simulink library "vmc"  (R2021b)
settings: Solver=VariableStepAuto  StartTime=0.0  StopTime=10.0  RelTol=1e-3
undefined symbols (not defined in the file or in its folder): AVMC_ACCDeltaTqIGain4OVRD_X_kph, AVMC_ACCDeltaTqIGain4OVRD_Y_mps2, AVMC_ACCDeltaTqIGain_X_kph, AVMC_ACCDeltaTqIGain_Y_mps2, AVMC_ACCDeltaTqPGain_X_kph, AVMC_ACCDeltaTqPGain_Y_kph, AVMC_ACCLongSteadyCtrl_X_kph, AVMC_ADSPosGFBDeltaTq_X_kph, AVMC_ADSPosGFBDeltaTq_Y_mps2, AVMC_AggressJerkPCT4AT_X_kph, AVMC_AggressJerkPCT_X_kph, AVMC_AggressLimitPCT4AT_X_kph, AVMC_AggressLimitPCT_X_kph, AVMC_CCLongSteadyCtrl_X_kph, AVMC_DISCDeltaTqIGain_X_kph, AVMC_DISCDeltaTqIGain_Y_mps2, AVMC_DISCDeltaTqPGain_X_kph, AVMC_DISCDeltaTqPGain_Y_kph, AVMC_ESCRegenOut_X_kph, AVMC_ESCRegenOut_Y_Deg, AVMC_ESCRegenOutEnSpd_X_Deg, AVMC_ISOAccLimit_X_mps, AVMC_ISODecLimit_X_mps, AVMC_ISOJerk_X_mps, AVMC_LatESCRegenOut_X_kph, AVMC_LatESCRegenOut_Y_Deg, AVMC_LongAccDeadZone_X_kph, AVMC_LongAccFiltTsforP2_X_Gps, AVMC_MCPresBaseTq_X_bar, AVMC_MSALongSteadyCtrl_X_kph, AVMC_MSAPedalOvrd_X_kph, AVMC_MSASpdBand_X_kph, AVMC_MSATqDownEndTq_X_kph, AVMC_MSATqDownTime_X_kph, AVMC_OPDDisSlideRate_X_Deg, AVMC_OVRD2ActSR2FCMCMD_X_mps2, AVMC_PedalTqRWhlRatio_X_Nm, AVMC_PedalTqRWhlRatio_Y_gps, AVMC_PedalTqRWhlSlipGain_X_rat, AVMC_PedalTqRWhlSlipGain_Y_kph, AVMC_PedalTqRWhSTRGGain_X_deg, AVMC_PedalTqRWhSTRGGain_Y_kph, AVMC_RDCDetectTime_X_kph, AVMC_RDCDetectTime_Y_pct, AVMC_RDCEnSlideRate_X_Deg, AVMC_RearWhlTqRatio_X_Nm, AVMC_RearWhlTqRatio_Y_gps, AVMC_RearWhlTqSlipGain_X_rat, AVMC_RearWhlTqSlipGain_Y_kph, AVMC_RearWhlTqSTRGGain_X_deg, AVMC_RearWhlTqSTRGGain_Y_kph, AVMC_ReqBrkJoinDecSR_X_mps2, AVMC_SoftJerkPCT_X_kph, AVMC_SoftLimitPCT_X_kph, AVMC_StESCYaw_X_kph, AVMC_StESCYaw_Y_Deg, AVMC_StESCYawCom_X_kph, AVMC_StESCYawCom_Y_Gps, AVMC_TMSpdBaseTq_X_rpm, AVMC_VehHoldDecCtrlTime2_X_kph ... (+405)
libraries: hcu_lib x105, simulink x75, tqr x1, simulink_extras x1
(part 2 of 14)

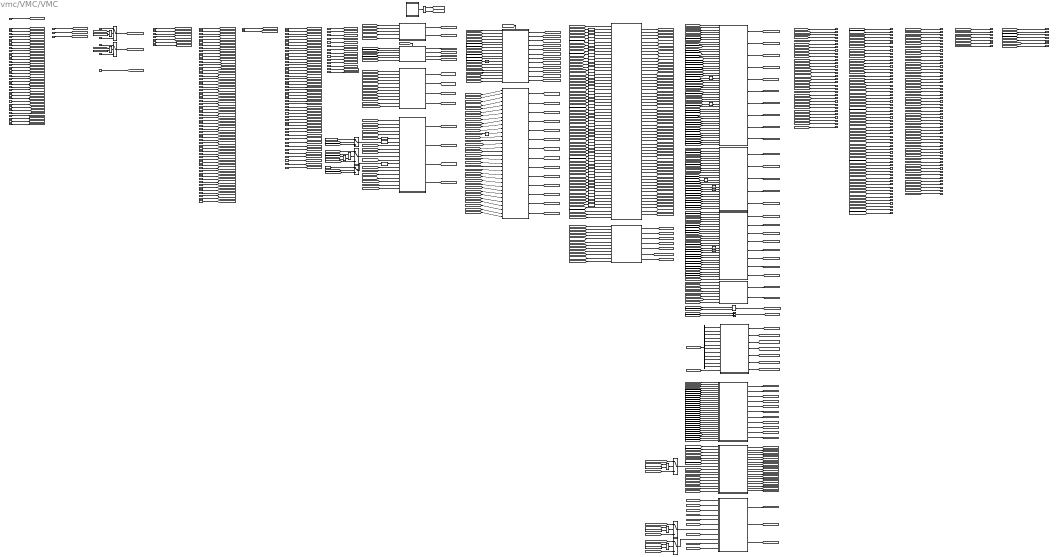
== system vmc/VMC/VMC ==
  note: AOICtrl
  note: VMC SW Version:
      | CR-No. B9 -> B10
      | Date: 2025/02/10
  note: Phase1_Add Functions for VCU
  note: FD
  note: GPIO
  note: CAN6
  note: DDM
  note: CAN3
  note: CAN2
  note: CAN1
  note: KPH2MPH_SetSpeed
  note: PreConditionCheck
  note: SPD2ACC
  note: VMC_FCM1
  note: SpeedArbitration
  note: ACC_CC_MSAWhlTq
  note: SafetyControl
  note: IMU
  note: SYS
  note: DSC
      | Test
      | Function
  note: For
      | DDM
      | 2024/12/21
  note: CAN4
  note: For
      | APS
      | 2025/02/07
  task_time_s : Inport
  VINP_DriverSeatBeltCmd_flg : Inport  Port=2
  VINP_MeterIndVehSpeed_kph : Inport  Port=3
  VINP_BrkSwSta_flg : Inport  Port=4
  VINP_EPBSta_enum : Inport  Port=5
  VINP_ACCAvail_flg : Inport  Port=6
  VINP_AEBAvail_flg : Inport  Port=7
  VINP_ESCOFFStatus_enum : Inport  Port=8
  VINP_VehSpeed_kph : Inport  Port=9
  VINP_LFRawWhlSpeed_kph : Inport  Port=10
  VINP_LFRawWhlSpeedV_flg : Inport  Port=11
  VINP_RFRawWhlSpeed_kph : Inport  Port=12
  VINP_RFRawWhlSpeedV_flg : Inport  Port=13
  VINP_LRRawWhlSpeed_kph : Inport  Port=14
  VINP_LRRawWhlSpeedV_flg : Inport  Port=15
  VINP_RRRawWhlSpeed_kph : Inport  Port=16
  VINP_RRRawWhlSpeedV_flg : Inport  Port=17
  VINP_LatAccel_Gps : Inport  Port=18
  VINP_LatAccelV_flg : Inport  Port=19
  VINP_GRADE_Deg : Inport  Port=20
  VINP_LongAccel_Gps : Inport  Port=21
  VINP_MCPressure_bar : Inport  Port=22
  VINP_ESCADASSta_enum : Inport  Port=23
  VINP_FrRBCActive_flg : Inport  Port=24
  VINP_RrRBCActive_flg : Inport  Port=25
  VINP_FrntAxlTrqReqBrk_Nm : Inport  Port=26
  VINP_RearAxlTrqReqBrk_Nm : Inport  Port=27
  VINP_BrkPedalPos_pct : Inport  Port=28
  VINP_SASAngle_Deg : Inport  Port=29
  VINP_ESCActive_flg : Inport  Port=30
  VINP_YawRate_degps : Inport  Port=31
  VINP_RDCActive_enum : Inport  Port=32
  VINP_LFWhlRotDir_enum : Inport  Port=33
  VINP_LRWhlRotDir_enum : Inport  Port=34
  VINP_RFWhlRotDir_enum : Inport  Port=35
  VINP_RRWhlRotDir_enum : Inport  Port=36
  VINP_Distanceunit_flg : Inport  Port=37
  VINP_IVISWCVibModeSta_enum : Inport  Port=38
  VINP_SmartEcoModeSW_flg : Inport  Port=39
  VINP_FrTMSpd_rpm : Inport  Port=40
  VINP_FrTMSpdNidec_rpm : Inport  Port=41
  VINP_RrTMSpd_rpm : Inport  Port=42
  VINP_RrTMSpdNidec_rpm : Inport  Port=43
  VINP_ADASAEBSta_enum : Inport  Port=44
  VINP_ADASACCSta_enum : Inport  Port=45
  VINP_ACCRequiredAccel_mps2 : Inport  Port=46
  VINP_ACCVehHoldReq_flg : Inport  Port=47
  VINP_ADASAEBReq_enum : Inport  Port=48
  VINP_ADASLKASta_enum : Inport  Port=49
  VINP_LKAStrToqReq_Nm : Inport  Port=50
  VINP_LKATOIFault_flg : Inport  Port=51
  VINP_LKATOIAct_enum : Inport  Port=52
  VINP_ADASFaultSta_flg : Inport  Port=53
  VINP_AEBVehHoldReq_flg : Inport  Port=54
  VINP_ADASDBSReq_enum : Inport  Port=55
  VINP_ACCObjDist_m : Inport  Port=56
  VINP_ACCObjRelSpd_mps : Inport  Port=57
  VINP_TimeGapLevel_enum : Inport  Port=58
  VINP_HazardWarningReq_flg : Inport  Port=59
  VINP_ADASForceIdle_flg : Inport  Port=60
  VINP_RightTurnLightReq_flg : Inport  Port=61
  VINP_LeftTurnLightReq_flg : Inport  Port=62
  VINP_ForceLowBeam_enum : Inport  Port=63
  VINP_ACCJerkUpperLimit_mps3 : Inport  Port=64
  VINP_ACCComfortBandUpper_mps2 : Inport  Port=65
  VINP_ACCJerkLowerLimit_mps3 : Inport  Port=66
  VINP_ACCComfortBandLower_mps2 : Inport  Port=67
  VINP_ADASVehSpdLim_raw32 : Inport  Port=68
  VINP_ADASShftPosnReqA_flg : Inport  Port=69
  VINP_ADASShftPosnReq_enum : Inport  Port=70
  VINP_ADASFCWSta_enum : Inport  Port=71
  VINP_ADASLDWSta_enum : Inport  Port=72
  VINP_ADASFltWrnReq_flg : Inport  Port=73
  VINP_ACCObjDstLvl_enum : Inport  Port=74
  VINP_ACCTakeoverReq_flg : Inport  Port=75
  VINP_ADASWarningMsg_enum : Inport  Port=76
  VINP_ADASCAMSpdLim_enum : Inport  Port=77
  VINP_TargetType_enum : Inport  Port=78
  VINP_ADASSLIFSpdLim_enum : Inport  Port=79
  VINP_LKAHODDisplayWarning_flg : Inport  Port=80
  VINP_LKAHODSoundWarning_flg : Inport  Port=81
  VINP_ADASLFCSta_enum : Inport  Port=82
  VINP_ADASLaneModeL_enum : Inport  Port=83
  VINP_ADASLaneModeR_enum : Inport  Port=84
  VINP_ADASSLIFSta_enum : Inport  Port=85
  VINP_ADASISASta_enum : Inport  Port=86
  VINP_ADASLDWMute_flg : Inport  Port=87
  VINP_ADASFCWMute_flg : Inport  Port=88
  VINP_ADASLFCHandsOffWarning_enum : Inport  Port=89
  VINP_LVDADisabled_flg : Inport  Port=90
  VINP_LVDAMuteSta_enum : Inport  Port=91
  VINP_LVDAFailinfo_flg : Inport  Port=92
  VINP_LVDAWarning_flg : Inport  Port=93
  VINP_LVDAACCStatusInformation_flg : Inport  Port=94
  VINP_ADASLFCWarnSound_enum : Inport  Port=95
  VINP_FCMACCmode_enum : Inport  Port=96
  VINP_ADASLanetypeR_enum : Inport  Port=97
  VINP_ADASLanetypeL_enum : Inport  Port=98
  VINP_ADASLanecurveL_raw32 : Inport  Port=99
  VINP_ADASLanecurveR_raw32 : Inport  Port=100
  VINP_ADASDrvInputTqBoostAct_flg : Inport  Port=101
  VINP_ADASStrWhlAngCtrlStatus_flg : Inport  Port=102
  VINP_ADASMaxAngCtrlOutTqLimit_Nm : Inport  Port=103
  VINP_ADASDrvInputTqBoostGain_pct : Inport  Port=104
  VINP_ADASAngCtrlTqWeightGain_pct : Inport  Port=105
  VINP_ADASDesStrWhlAngCtrlCmd_Deg : Inport  Port=106
  VINP_BrakeSWGPIO_flg : Inport  Port=107
  VINP_HoodSW_flg : Inport  Port=108
  APP_SpdLimit_flg : Inport  Port=109
  APP_SpdLimit : Inport  Port=110
  VINP_DIDGetDynoMode_flg : Inport  Port=111
  VINP_VehicleType_enum : Inport  Port=112
  VINP_SWCType_enum : Inport  Port=113
  VINP_APSStaSystem_enum : Inport  Port=114
  VINP_APSDecReqA_flg : Inport  Port=115
  VINP_APSDecReq_mps2 : Inport  Port=116
  VINP_APSReq_enum : Inport  Port=117
  VINP_APSShiftPosnReq_enum : Inport  Port=118
  VINP_APSSpeedCMD_kph : Inport  Port=119
  VINP_APSVMCReqA_flg : Inport  Port=120
  VINP_CAASVMCReqA_flg : Inport  Port=121
  VINP_APSVRqEPASCtrl_flg : Inport  Port=122
  VINP_APSRqEPASCtrl_flg : Inport  Port=123
  VINP_APSAngleTarget_Deg : Inport  Port=124
  VBCM_DrDoorSW_flg : Inport  Port=125
  VDSC_DISCTurn_flg : Inport  Port=126
  VDSC_DISCSta_enum : Inport  Port=127
  VDSC_DISCTargetSpd_kph : Inport  Port=128
  VDSC_TurningSpdMovingflat_kph : Inport  Port=129
  VDSC_AutoTurnMode_flg : Inport  Port=130
  VDSC_AccDecResp_flg : Inport  Port=131
  VDSC_PreACC_flg : Inport  Port=132
  VDSC_PreACC_mps2 : Inport  Port=133
  VTQD_DriverWhlTqDem_Nm : Inport  Port=134
  VTQD_CoordWhlTqDemFr_Nm : Inport  Port=135
  VTQD_CoordWhlTqDemRr_Nm : Inport  Port=136
  VTQD_GearActualPosn_enum : Inport  Port=137
  VTQD_ExternalTqAllow_flg : Inport  Port=138
  VTQD_LowIdleAccPedal_flg : Inport  Port=139
  VTQD_ExtShftAllow_flg : Inport  Port=140
  VTQD_FrEDUAvailBrkRgnTq_Nm : Inport  Port=141
  VTQD_RrEDUAvailBrkRgnTq_Nm : Inport  Port=142
  VTQD_APSStaSys_enum : Inport  Port=143
  VTQD_APSDecReqA_flg : Inport  Port=144
  VTQD_APSDecReq_mps2 : Inport  Port=145
  VTQD_APSReq_enum : Inport  Port=146
  VTQD_AfterAvailableTqDemFr_Nm : Inport  Port=147
  VTQD_AfterAvailableTqDemRr_Nm : Inport  Port=148
  VTQD_EquivAccPedalSWSta_flg : Inport  Port=149
  VTQD_ExtDoorAllow_flg : Inport  Port=150
  VTQD_SpdCtrlSta_flg : Inport  Port=151
  VTQD_SpdCtrlMode_enum : Inport  Port=152
  VTQD_RegenMode_enum : Inport  Port=153
  VTQD_SetSpd_kph : Inport  Port=154
  VTQD_SWC2ResUpSta_flg : Inport  Port=155
  VTQD_SWC2SetdownSta_flg : Inport  Port=156
  VTQD_SWC2CANCELSta_flg : Inport  Port=157
  VTQD_CreepBaseTqD_Nm : Inport  Port=158
  VTQD_VehActSpd_kph : Inport  Port=159
  VTQD_EVDriveMode_enum : Inport  Port=160
  VTQD_SWC1CANCELSta_flg : Inport  Port=161
  VTQD_SWC1ResUpSta_flg : Inport  Port=162
  VTQD_SWC1SetdownSta_flg : Inport  Port=163
  VTQD_EPBCarWashMode_flg : Inport  Port=164
  VTQR_RrTMTqReq_Nm : Inport  Port=165
  VTQR_FrTMTqReq_Nm : Inport  Port=166
  VDHP_ActAPSPosn_pct : Inport  Port=167
  <VPMM_DrivetrainSelect_enum> : Inport  Port=168
  BINP_IMU_outputs : Inport  Port=169  OutDataTypeStr=Bus: BINP_IMU_outputs
  VDDM_VMCLongCtrlProhibited_flg : Inport  Port=170
  VDDM_VMCLatCtrlProhibited_flg : Inport  Port=171
  VDDM_VMCESC1Err_flg : Inport  Port=172
  VDDM_VMCESC5Err_flg : Inport  Port=173
  VDDM_VMCEPSErr_flg : Inport  Port=174
  VDDM_VCURAPSErrLv2_flg : Inport  Port=175
  VDDM_VCURAPSErrLv3_flg : Inport  Port=176
  VINP_SCPSystemMode_enum : Inport  Port=177
  ACC_Function : Subsystem
  AND{4..6,9} (4 alike) : Logic  AllPortsSameDT=off  OutDataTypeStr=boolean
  APS function : Subsystem
  Add : Sum
  Bus Selector10 : BusSelector  OutputSignals=VINP_MemOffsetGyroX_raw16,VINP_MemOffsetGyroY_raw16,VINP_MemOffsetGyroZ_raw16,VINP_MemOffsetAccX_raw16,VINP_MemOffsetAccY_raw16,VINP_MemOffsetAccZ_raw16,VINP_SensingGyroX_raw16,VINP_SensingGyroY_raw16,VINP_SensingGyroZ_raw16,VINP_SensingAccX_raw16,VINP_SensingAccY_raw16,VINP_SensingAccZ_raw16
  Cast To Single{1,7,12,17,19..20,22,25..26,28..31,33..34,36,38..40,43..47,50,52,56..59,62} (31 alike) : DataTypeConversion  OutDataTypeStr=uint8
  Cast To Single{3..6,8..10,18,60..61} (10 alike) : DataTypeConversion  OutDataTypeStr=single
  Cast To Single{2,11,13..16,21,23..24,27,37,41..42,48..49,51,53..55} (19 alike) : DataTypeConversion  OutDataTypeStr=boolean
  Constant10 : Constant  Value=KVMC_RDCRzSource_flg
  Constant109 : Constant  Value=TRUE
  Constant11 : Constant  Value=KVMC_SlideRateGxSource_flg
  Constant14 : Constant  Value=ENUM_VEHICLETYPE_D31L24
  Constant15 : Constant  Value=ENUM_DISCSTA_ACTIVE
  Constant28 : Constant  Value=KVMC_RDCGySource_flg
  Constant6 : Constant  Value=ENUM_VEHICLETYPE_D31L24
  Constant7 : Constant  Value=ENUM_DISCSTA_ACTIVE
  CruiseControlFunction : Subsystem
  Equal1 : RelationalOperator  Operator=~=  OutDataTypeStr=boolean  RndMeth=Simplest
  Equal2 : RelationalOperator  Operator=~=  OutDataTypeStr=boolean  RndMeth=Simplest
  FeatureSetSpeed : Subsystem
  Function-Call Split : FunctionCallSplit  IconShape=distinctive  NumOutputPorts=2  OutputPortLayout=default
  IMU : Subsystem
  LFCAOIControl : Subsystem
  Logical Operator : Logic  Operator=OR  AllPortsSameDT=off  OutDataTypeStr=boolean
  Long Acceleration Calculation : Subsystem
  MSA function : Subsystem
  PreConditionCheck : Subsystem
  RDC Determination : Subsystem
  Relational Operator8 : RelationalOperator  Operator=~=  OutDataTypeStr=boolean  RndMeth=Simplest
  SPD2ACC : Subsystem
  SafetyControl : Subsystem  TreatAsAtomicUnit=on
  Scheduler : Stateflow chart  TreatAsAtomicUnit=on
  Slide Rate  Calculation : Subsystem
  SpeedArbitration : Subsystem
  SpeedCalculation : Subsystem  TreatAsAtomicUnit=on
  Switch{1..8} (8 alike) : Switch  Criteria=u2 > Threshold
  Unit Delay{,1..2,5..8} (7 alike) : UnitDelay  SampleTime=-1  HasFrameUpgradeWarning=on
  VMC_FCM1 : Subsystem
  initial = 0 : UnitDelay  SampleTime=-1  HasFrameUpgradeWarning=on
  VVMC_FeatSetSpdFinal_raw32 : Outport
  VVMC_VehicleSpeed_mph : Outport  Port=2
  VVMC_VehicleSpeed_kph : Outport  Port=3
  VVMC_MeterIndSpeed_raw32 : Outport  Port=4
  VVMC_MeterIndSpeedForCalcu_kph : Outport  Port=5
  VVMC_VMCAEBCtrlAvail_flg : Outport  Port=6
  VVMC_VMCACCCtrlAvail_flg : Outport  Port=7
  VVMC_VMCCCCtrlAvail_flg : Outport  Port=8
  VVMC_VMCMSACtrlAvail_flg : Outport  Port=9
  VVMC_FeatArbitrSta_enum : Outport  Port=10
  VVMC_FeatReqSpd_kph : Outport  Port=11
  VVMC_JerkPCT_pct : Outport  Port=12
  VVMC_LimitPCT_pct : Outport  Port=13
  VVMC_LFWhlSpeedRollAve_kph : Outport  Port=14
  VVMC_RFWhlSpeedRollAve_kph : Outport  Port=15
  VVMC_LRWhlSpeedRollAve_kph : Outport  Port=16
  VVMC_RRWhlSpeedRollAve_kph : Outport  Port=17
  VVMC_FrontRearSlipRatioCtrl_flg : Outport  Port=18
  VVMC_RearWhlSlipRatioCtrl_flg : Outport  Port=19
  VVMC_SingleWhlSlipRatioCtrl_flg : Outport  Port=20
  VVMC_LatAccCtrl_flg : Outport  Port=21
  VVMC_SafetyCtrl_flg : Outport  Port=22
  VVMC_EstSlope_Deg : Outport  Port=23
  VVMC_SPD2ACCAct_flg : Outport  Port=24
  VVMC_AccCalcuPID_mps2 : Outport  Port=25
  VVMC_ISOAccLimit_mps2 : Outport  Port=26
  VVMC_ISODecLimit_mps2 : Outport  Port=27
  VVMC_ISOJerkLimit_mps3 : Outport  Port=28
  VVMC_ACCRequiredAccel_mps2 : Outport  Port=29
  VVMC_DISCReqAcc_mps2 : Outport  Port=30
  VVMC_FeatArbitrFinal_enum : Outport  Port=31
  VVMC_ActACCRequiredAccel_mps2 : Outport  Port=32
  VVMC_LateralCtrl_flg : Outport  Port=33
  VVMC_ADASLKASta_enum : Outport  Port=34
  VVMC_LKAStrToqReq_Nm : Outport  Port=35
  VVMC_LKATOIFault_flg : Outport  Port=36
  VVMC_LKATOIAct_enum : Outport  Port=37
  VVMC_ADASAEBReq_enum : Outport  Port=38
  VVMC_ADASFaultSta_flg : Outport  Port=39
  VVMC_AEBVehHoldReq_flg : Outport  Port=40
  VVMC_ACCVehHoldReq_flg : Outport  Port=41
  VVMC_ADASDBSReq_enum : Outport  Port=42
  VVMC_ADASACCSta_enum : Outport  Port=43
  VVMC_ACCObjDist_m : Outport  Port=44
  VVMC_ACCObjRelSpd_mps : Outport  Port=45
  VVMC_TimeGapLevel_enum : Outport  Port=46
  VVMC_ACCJerkUpperLimit_mps3 : Outport  Port=47
  VVMC_ACCComfortBandUpper_mps2 : Outport  Port=48
  VVMC_ACCJerkLowerLimit_mps3 : Outport  Port=49
  VVMC_ACCComfortBandLower_mps2 : Outport  Port=50
  VVMC_ADASVehSpdLim_raw32 : Outport  Port=51
  VVMC_ADASShftPosnReqA_flg : Outport  Port=52
  VVMC_ADASShftPosnReq_enum : Outport  Port=53
  VVMC_ADASForceIdle_flg : Outport  Port=54
  VVMC_HazardWarningReq_flg : Outport  Port=55
  VVMC_RightTurnLightReq_flg : Outport  Port=56
  VVMC_LeftTurnLightReq_flg : Outport  Port=57
  VVMC_ADASFCWSta_enum : Outport  Port=58
  VVMC_ADASLDWSta_enum : Outport  Port=59
  VVMC_ADASFltWrnReq_flg : Outport  Port=60
  VVMC_ACCObjDstLvl_enum : Outport  Port=61
  VVMC_ForceLowBeam_enum : Outport  Port=62
  VVMC_ACCTakeoverReq_flg : Outport  Port=63
  VVMC_ADASWarningMsg_enum : Outport  Port=64
  VVMC_ADASCAMSpdLim_enum : Outport  Port=65
  VVMC_TargetType_enum : Outport  Port=66
  VVMC_ADASSLIFSpdLim_enum : Outport  Port=67
  VVMC_LKAHODDisplayWarning_flg : Outport  Port=68
  VVMC_LKAHODSoundWarning_flg : Outport  Port=69
  VVMC_ADASLFCSta_enum : Outport  Port=70
  VVMC_ADASLaneModeL_enum : Outport  Port=71
  VVMC_ADASLaneModeR_enum : Outport  Port=72
  VVMC_ADASSLIFSta_enum : Outport  Port=73
  VVMC_ADASISASta_enum : Outport  Port=74
  VVMC_ADASLDWMute_flg : Outport  Port=75
  VVMC_ADASFCWMute_flg : Outport  Port=76
  VVMC_ADASLFCHandsOffWarning_enum : Outport  Port=77
  VVMC_LVDADisabled_flg : Outport  Port=78
  VVMC_LVDAMuteSta_enum : Outport  Port=79
  VVMC_LVDAFailinfo_flg : Outport  Port=80
  VVMC_LVDAWarning_flg : Outport  Port=81
  VVMC_LVDAACCStatusInformation_flg : Outport  Port=82
  VVMC_ADASLFCWarnSound_enum : Outport  Port=83
  VVMC_FCMACCmode_enum : Outport  Port=84
  VVMC_ADASLanetypeR_enum : Outport  Port=85
  VVMC_ADASLanetypeL_enum : Outport  Port=86
  VVMC_ADASLanecurveL_raw32 : Outport  Port=87
  VVMC_ADASLanecurveR_raw32 : Outport  Port=88
  VVMC_ADASAEBSta_enum : Outport  Port=89
  VVMC_FCMLDWRequest_enum : Outport  Port=90
  VVMC_FCMLDWFault_flg : Outport  Port=91
  VVMC_ADASActive_flg : Outport  Port=92
  VVMC_ACCCtrlAvail_flg : Outport  Port=93
  VVMC_ADASNegReq_flg : Outport  Port=94
  VVMC_ACCPedalOvrd_flg : Outport  Port=95
  VVMC_ADASWhlTqReq_Nm : Outport  Port=96
  VVMC_AccPedalOvrdDISC_flg : Outport  Port=97
  VVMC_RearTqRatio_rat : Outport  Port=98
  VVMC_TimeGapCalcu_s : Outport  Port=99
  VVMC_CCCtrlSta_enum : Outport  Port=100
  VVMC_CruzActive_flg : Outport  Port=101
  VVMC_CCPedalOvrd_flg : Outport  Port=102
  VVMC_CruzWhlTqReq_Nm : Outport  Port=103
  VVMC_MSACtrlSta_enum : Outport  Port=104
  VVMC_MSAActive_flg : Outport  Port=105
  VVMC_MSAWhlTqReq_Nm : Outport  Port=106
  VVMC_APSCtrlAvail_flg : Outport  Port=107
  VVMC_APSActive_flg : Outport  Port=108
  VVMC_APSSpeedCMD_kph : Outport  Port=109
  VVMC_APSShiftPosnReq_enum : Outport  Port=110
  VVMC_APSStaSys_enum : Outport  Port=111
  VVMC_APSDecReqA_flg : Outport  Port=112
  VVMC_APSDecReq_mps2 : Outport  Port=113
  VVMC_APSReq_enum : Outport  Port=114
  VVMC_LongAcc_Gps : Outport  Port=115
  VVMC_RawWhlSpdSlideRate_pct : Outport  Port=116
  VVMC_LFWhlSpdSlideRate_pct : Outport  Port=117
  VVMC_RFWhlSpdSlideRate_pct : Outport  Port=118
  VVMC_LRWhlSpdSlideRate_pct : Outport  Port=119
  VVMC_RRWhlSpdSlideRate_pct : Outport  Port=120
  VVMC_PredictVehSpd_kph : Outport  Port=121
  VVMC_LF4WhlSpdSlideRate_pct : Outport  Port=122
  VVMC_RF4WhlSpdSlideRate_pct : Outport  Port=123
  VVMC_LR4WhlSpdSlideRate_pct : Outport  Port=124
  VVMC_RR4WhlSpdSlideRate_pct : Outport  Port=125
  VVMC_4WhlSpdSlideRate_pct : Outport  Port=126
  VVMC_ActMaxSlideRate_pct : Outport  Port=127
  VVMC_ActLFSlideRate_pct : Outport  Port=128
  VVMC_ActRFSlideRate_pct : Outport  Port=129
  VVMC_ActLRSlideRate_pct : Outport  Port=130
  VVMC_ActRRSlideRate_pct : Outport  Port=131
  VVMC_AltLWhlSlideRate_pct : Outport  Port=132
  VVMC_AltRWhlSlideRate_pct : Outport  Port=133
  VVMC_AltWhlSlideRate_pct : Outport  Port=134
  VVMC_CCMSASpdWar_flg : Outport  Port=135
  VVMC_IMUEnaCmd_flg : Outport  Port=136
  VVMC_RWDRDCActive_enum : Outport  Port=137
  VVMC_MSAWhlTqActive_flg : Outport  Port=138
  VVMC_RDCEnSlideRate_pct : Outport  Port=139
  VVMC_ActStESCYaw_Dps : Outport  Port=140
  VVMC_ACCOvrdMemTq_Nm : Outport  Port=141
  VVMC_CAASCtrlAvail_flg : Outport  Port=142
  VVMC_CAASActive_flg : Outport  Port=143
  "VVMC_ExtraMSACtrlSta_enum " : Outport  Port=144
  VVMC_CalibratedAccX_G : Outport  Port=145
  VVMC_CalibratedAccY_G : Outport  Port=146
  VVMC_CalibratedAccZ_G : Outport  Port=147
  VVMC_CalibratedGyroX_Dps : Outport  Port=148
  VVMC_CalibratedGyroY_Dps : Outport  Port=149
  VVMC_CalibratedGyroZ_Dps : Outport  Port=150
  VVMC_SetACCDisableAPS_flg : Outport  Port=151
  VVMC_FDCVMCAPSVRqEPSCtrl_flg : Outport  Port=152
  VVMC_FDCVMCAPSAngleTarget_deg : Outport  Port=153
  VVMC_FDCVMCAPSRqEPSCtrl_flg : Outport  Port=154
  VVMC_FDCVMCAngCtrlTqWtGn_pct : Outport  Port=155
  VVMC_FDCVMCDrInpTqBstAct_flg : Outport  Port=156
  VVMC_FDCVMCMaxAngCtrlOutTqLim_Nm : Outport  Port=157
  VVMC_FDCVMCDrInpTqBstGn_pct : Outport  Port=158
  wires:
  [VINP_VehSpeed_kph] -> SpeedArbitration/15(VINP_VehSpeed_kph)
  [VVMC_MeterIndSpeedForCalcu_kph] -> SpeedArbitration/14(VVMC_MeterIndSpeedForCalcu_kph)
  [VVMC_FeatArbitrFinal_enum] -> initial = 0/1
  [task_time_s] -> SPD2ACC/10(task_time_s)
  SpeedCalculation/4(VVMC_MeterIndSpeedForCalcu_kph) -> [VVMC_MeterIndSpeedForCalcu_kph]
  [VVMC_FeatReqSpd_kph] -> ACC_Function/19(VVMC_FeatReqSpd_kph)
  [task_time_s] -> PreConditionCheck/11(task_time_s)
  SpeedCalculation/3(VVMC_VehicleSpeed_kph) -> [VVMC_VehicleSpeed_kph]
  SpeedCalculation/2(VVMC_VehicleSpeed_mph) -> [VVMC_VehicleSpeed_mph]
  [VINP_VehSpeed_kph] -> Long Acceleration Calculation/3(VINP_VehSpeed_kph)
  [VINP_ESCADASSta_enum] -> ACC_Function/18(VINP_ESCADASSta_enum)  "VINP_ESCADASSta_enum"
  [VINP_MCPressure_bar] -> ACC_Function/17(VINP_MCPressure_bar)  "VINP_MCPressure_bar"
  [VINP_RrTMSpd_rpm] -> ACC_Function/16(VINP_RrTMSpd_rpm)  "VINP_RrTMSpd_rpm"
  [VINP_FrTMSpd_rpm] -> ACC_Function/15(VINP_FrTMSpd_rpm)  "VINP_FrTMSpd_rpm"
  VINP_FrRBCActive_flg/1 -> [VINP_FrRBCActive_flg]
  VINP_RrRBCActive_flg/1 -> [VINP_RrRBCActive_flg]
  VTQD_RegenMode_enum/1 -> [VTQD_RegenMode_enum]
  VINP_ESCADASSta_enum/1 -> [VINP_ESCADASSta_enum]
  VINP_MCPressure_bar/1 -> [VINP_MCPressure_bar]
  VINP_RrTMSpdNidec_rpm/1 -> Switch3/3
  [VINP_VehSpeed_kph] -> SPD2ACC/6(VINP_VehSpeed_kph)
  VINP_Distanceunit_flg/1 -> [VINP_Distanceunit_flg]
  [VINP_ADASACCSta_enum] -> SpeedArbitration/8(VINP_ADASACCSta_enum)  "VINP_ADASACCSta_enum"
  SPD2ACC/3(VVMC_FeatArbitrFinal_enum) -> [VVMC_FeatArbitrFinal_enum]
  [VINP_ACCObjDist_m] -> ACC_Function/12(VINP_ACCObjDist_m)  "VINP_ACCObjDist_m"
  ACC_Function/3(VVMC_ADASWhlTqReq_Nm) -> [VVMC_ADASWhlTqReq_Nm]
  [VTQD_CoordWhlTqDemFr_Nm] -> ACC_Function/4(VTQD_CoordWhlTqDemFr_Nm)  "VTQD_CoordWhlTqDemFr_Nm"
  [task_time_s] -> ACC_Function/1(task_time_s)  "task_time_s"
  SpeedArbitration/4(VVMC_LimitPCT_pct) -> [VVMC_LimitPCT_pct]
  [VTQD_ExternalTqAllow_flg] -> ACC_Function/3(VTQD_ExternalTqAllow_flg)  "VTQD_ExternalTqAllow_flg"
  [VINP_VehSpeed_kph] -> ACC_Function/7(VINP_VehSpeed_kph)
  SpeedArbitration/3(VVMC_JerkPCT_pct) -> [VVMC_JerkPCT_pct]
  [VVMC_VMCMSACtrlAvail_flg] -> SpeedArbitration/2(VVMC_VMCMSACtrlAvail_flg)
  [VINP_TimeGapLevel_enum] -> ACC_Function/14(VINP_TimeGapLevel_enum)  "VINP_TimeGapLevel_enum"
  [VVMC_FeatReqSpd_kph] -> SPD2ACC/3(VVMC_FeatReqSpd_kph)
  CruiseControlFunction/4(VVMC_CruzActive_flg) -> [VVMC_CruzActive_flg]
  CruiseControlFunction/2(VVMC_CCSpdWar_flg) -> [VVMC_CCSpdWar_flg]
  [VINP_LKATOIFault_flg] -> Cast To Single21/1
  [VTQD_SpdCtrlSta_flg] -> FeatureSetSpeed/2(VTQD_SpdCtrlSta_flg)  "VTQD_SpdCtrlSta_flg"
  Cast To Single20/1 -> VMC_FCM1/5(VINP_LKATOIAct_enum)  "VINP_LKATOIAct_enum"
  [VVMC_FeatSetSpdForCalcu_kph] -> CruiseControlFunction/12(VVMC_FeatSetSpdForCalcu_kph)
  [VVMC_MSACtrlSta_enum] -> SpeedArbitration/10(VVMC_MSACtrlSta_enum)  "VVMC_MSACtrlSta_enum"
  [VINP_DriverSeatBeltCmd_flg] -> PreConditionCheck/1(VINP_DriverSeatBeltCmd_flg)  "VINP_DriverSeatBeltCmd_flg"
  SpeedCalculation/1(VVMC_MeterIndSpeed_raw32) -> [VVMC_MeterIndSpeed_raw32]
  [VTQD_SetSpd_kph] -> FeatureSetSpeed/4(VTQD_SetSpd_kph)  "VTQD_SetSpd_kph"
  MSA function/3(VVMC_MSASpdWar_flg) -> [VVMC_MSASpdWar_flg]
  PreConditionCheck/4(VVMC_VMCMSACtrlAvail_flg) -> [VVMC_VMCMSACtrlAvail_flg]
  [VTQD_GearActualPosn_enum] -> PreConditionCheck/3(VTQD_GearActualPosn_enum)  "VTQD_GearActualPosn_enum"
  [VVMC_SafetyCtrl_flg] -> SPD2ACC/8(VVMC_SafetyCtrl_flg)  "VVMC_SafetyCtrl_flg"
  Cast To Single25/1 -> VMC_FCM1/10(VINP_ADASDBSReq_enum)  "VINP_ADASDBSReq_enum"
  CruiseControlFunction/1(VVMC_CCCtrlSta_enum) -> [VVMC_CCCtrlSta_enum]
  ACC_Function/1(VVMC_ACCCtrlAvail_flg) -> [VVMC_ACCCtrlAvail_flg]
  MSA function/4(VVMC_MSAActive_flg) -> [VVMC_MSAActive_flg]
  [VTQD_DriverWhlTqDem_Nm] -> MSA function/2(VTQD_DriverWhlTqDem_Nm)  "VTQD_DriverWhlTqDem_Nm"
  Logical Operator/1 -> [VVMC_CCMSASpdWar_flg]  "VVMC_CCMSASpdWar_flg"
  [VVMC_ActACCRequiredAccel_mps2] -> ACC_Function/10(VVMC_ActACCRequiredAccel_mps2)
  [VVMC_LongAcc_Gps] -> CruiseControlFunction/11(VVMC_LongAcc_Gps)
  ACC_Function/4(VVMC_ADASActive_flg) -> [VVMC_ADASActive_flg]
  [VINP_ADASAEBSta_enum] -> Cast To Single33/1
  [VTQD_ExternalTqAllow_flg] -> PreConditionCheck/9(VTQD_ExternalTqAllow_flg)  "VTQD_ExternalTqAllow_flg"
  [APP_SpdLimit_flg] -> FeatureSetSpeed/1(APP_SpdLimit_flg)  "APP_SpdLimit_flg"
  [VINP_APSStaSystem_enum] -> PreConditionCheck/8(VINP_APSStaSystem_enum)  "VINP_APSStaSystem_enum"
  PreConditionCheck/2(VVMC_VMCAEBCtrlAvail_flg) -> [VVMC_VMCAEBCtrlAvail_flg]
  FeatureSetSpeed/1(VVMC_FeatSetSpdFinal_raw32) -> [VVMC_FeatSetSpdFinal_raw32]
  [VINP_ACCAvail_flg] -> PreConditionCheck/5(VINP_ACCAvail_flg)  "VINP_ACCAvail_flg"
  SPD2ACC/1(VVMC_ACCRequiredAccel_mps2) -> [VVMC_ACCRequiredAccel_mps2]
  [VTQD_SpdCtrlMode_enum] -> CruiseControlFunction/4(<VTQD_SpdCtrlMode_enum>)  "VTQD_SpdCtrlMode_enum"
  [VVMC_MeterIndSpeedForCalcu_kph] -> SPD2ACC/7(VVMC_MeterIndSpeedForCalcu_kph)
  [VINP_ADASACCSta_enum] -> SPD2ACC/2(VINP_ADASACCSta_enum)  "VINP_ADASACCSta_enum"
  [VINP_ACCRequiredAccel_mps2] -> SPD2ACC/9(VINP_ACCRequiredAccel_mps2)  "VINP_ACCRequiredAccel_mps2"
  SPD2ACC/2(VVMC_DISCReqAcc_mps2) -> [VVMC_DISCReqAcc_mps2]  "VVMC_DISCReqAcc_mps2"
  [VDSC_DISCSta_enum] -> Switch4/3
  Cast To Single22/1 -> VMC_FCM1/6(VINP_ADASAEBReq_enum)  "VINP_ADASAEBReq_enum"
  [VINP_ACCVehHoldReq_flg] -> Cast To Single2/1
  [VVMC_FeatArbitrSta_enum] -> SPD2ACC/1(VVMC_FeatArbitrSta_enum)
  [VINP_LKATOIAct_enum] -> Cast To Single20/1
  Cast To Single24/1 -> VMC_FCM1/8(VINP_AEBVehHoldReq_flg)  "VINP_AEBVehHoldReq_flg"
  [VINP_AEBVehHoldReq_flg] -> Cast To Single24/1
  Cast To Single18/1 -> VMC_FCM1/3(VINP_LKAStrToqReq_Nm)  "VINP_LKAStrToqReq_Nm"
  [VINP_ADASDBSReq_enum] -> Cast To Single25/1
  [VINP_ADASLKASta_enum] -> Cast To Single19/1
  [VVMC_FeatArbitrFinal_enum] -> VMC_FCM1/1(VVMC_FeatArbitrFinal_enum)
  [VINP_ADASFaultSta_flg] -> Cast To Single23/1
  [VTQD_DriverWhlTqDem_Nm] -> ACC_Function/2(VTQD_DriverWhlTqDem_Nm)  "VTQD_DriverWhlTqDem_Nm"
  [VVMC_FeatSetSpdForCalcu_kph] -> SpeedArbitration/12(VVMC_FeatSetSpdForCalcu_kph)
  Cast To Single28/1 -> VMC_FCM1/11(VINP_ADASACCSta_enum)  "VINP_ADASACCSta_enum"
  [VINP_EPBSta_enum] -> PreConditionCheck/4(VINP_EPBSta_enum)  "VINP_EPBSta_enum"
  SpeedArbitration/1(VVMC_FeatArbitrSta_enum) -> [VVMC_FeatArbitrSta_enum]
  [VTQD_LowIdleAccPedal_flg] -> ACC_Function/6(VTQD_LowIdleAccPedal_flg)  "VTQD_LowIdleAccPedal_flg"
  [VVMC_MSASpdWar_flg] -> Logical Operator/2
  [VINP_LKAStrToqReq_Nm] -> Cast To Single18/1
  Long Acceleration Calculation/1(VVMC_LongAcc_Gps) -> [VVMC_LongAcc_Gps]
  CruiseControlFunction/3(VVMC_CruzWhlTqReq_Nm) -> [VVMC_CruzWhlTqReq_Nm]
  [VTQD_ExternalTqAllow_flg] -> MSA function/1(VTQD_ExternalTqAllow_flg)  "VTQD_ExternalTqAllow_flg"
  [VINP_BrkSwSta_flg] -> CruiseControlFunction/9(VINP_BrkSwSta_flg)  "VINP_BrkSwSta_flg"
  Cast To Single23/1 -> VMC_FCM1/7(VINP_ADASFaultSta_flg)  "VINP_ADASFaultSta_flg"
  [VINP_VehSpeed_kph] -> MSA function/5(VINP_VehSpeed_kph)
  PreConditionCheck/1(VVMC_VMCACCCtrlAvail_flg) -> [VVMC_VMCACCCtrlAvail_flg]
  [VINP_BrakeSWGPIO_flg] -> CruiseControlFunction/8(VINP_BrakeSWGPIO_flg)  "VINP_BrakeSWGPIO_flg"
  [VTQD_SWC1CANCELSta_flg] -> CruiseControlFunction/7(VTQD_SWC1CANCELSta_flg)  "VTQD_SWC1CANCELSta_flg"
  Cast To Single33/1 -> SpeedArbitration/6(VINP_ADASAEBSta_enum)  "VINP_ADASAEBSta_enum"
  Cast To Single34/1 -> SpeedArbitration/13(VDSC_DISCTurn_flg)  "VDSC_DISCTurn_flg"
  [VINP_GRADE_Deg] -> Long Acceleration Calculation/1(VINP_GRADE_Deg)  "VINP_GRADE_Deg"
  [VTQD_CoordWhlTqDemRr_Nm] -> ACC_Function/5(VTQD_CoordWhlTqDemRr_Nm)  "VTQD_CoordWhlTqDemRr_Nm"
  Cast To Single7/1 -> CruiseControlFunction/14(VINP_ADASAEBSta_enum)  "VINP_ADASAEBSta_enum"
  [VINP_ADASAEBReq_enum] -> SpeedArbitration/5(VINP_ADASAEBReq_enum)  "VINP_ADASAEBReq_enum"
  ACC_Function/5(VVMC_TimeGapCalcu_s) -> [VVMC_TimeGapCalcu_s]
  [VBCM_DrDoorSW_flg] -> PreConditionCheck/2(VBCM_DrDoorSW_flg)  "VBCM_DrDoorSW_flg"
  [VVMC_LongAcc_Gps] -> ACC_Function/8(VVMC_LongAcc_Gps)
  [VINP_AEBAvail_flg] -> PreConditionCheck/6(VINP_AEBAvail_flg)  "VINP_AEBAvail_flg"
  [VTQD_SpdCtrlMode_enum] -> MSA function/3(<VTQD_SpdCtrlMode_enum>)  "VTQD_SpdCtrlMode_enum"
  [VINP_ADASAEBSta_enum] -> Cast To Single7/1
  [VINP_VehSpeed_kph] -> CruiseControlFunction/10(VINP_VehSpeed_kph)
  [VVMC_FeatArbitrFinal_enum] -> CruiseControlFunction/13(VVMC_FeatArbitrFinal_enum)
  SpeedArbitration/2(VVMC_FeatReqSpd_kph) -> [VVMC_FeatReqSpd_kph]
  [VVMC_LimitPCT_pct] -> SPD2ACC/4(VVMC_LimitPCT_pct)
  [VVMC_VMCCCCtrlAvail_flg] -> SpeedArbitration/1(VVMC_VMCCCCtrlAvail_flg)
  [VTQD_SWC1SetdownSta_flg] -> CruiseControlFunction/6(VTQD_SWC1SetdownSta_flg)  "VTQD_SWC1SetdownSta_flg"
  [VTQD_SWC2SetdownSta_flg] -> MSA function/10(VTQD_SWC2SetdownSta_flg)  "VTQD_SWC2SetdownSta_flg"
  [VINP_ADASACCSta_enum] -> Cast To Single28/1
  Cast To Single2/1 -> VMC_FCM1/9(VINP_ACCVehHoldReq_flg)  "VINP_ACCVehHoldReq_flg"
  Cast To Single31/1 -> SpeedArbitration/7(VDSC_DISCSta_enum)  "VDSC_DISCSta_enum"
  [VINP_LongAccel_Gps] -> Long Acceleration Calculation/2(VINP_LongAccel_Gps)  "VINP_LongAccel_Gps"
  [APP_SpdLimit] -> FeatureSetSpeed/3(APP_SpdLimit)  "APP_SpdLimit"
  [VINP_ESCOFFStatus_enum] -> PreConditionCheck/7(VINP_ESCOFFStatus_enum)  "VINP_ESCOFFStatus_enum"
  [VTQD_SWC2ResUpSta_flg] -> MSA function/9(VTQD_SWC2ResUpSta_flg)  "VTQD_SWC2ResUpSta_flg"
  [VVMC_FeatSetSpdForCalcu_kph] -> ACC_Function/11(VVMC_FeatSetSpdForCalcu_kph)
  [VVMC_MeterIndSpeedForCalcu_kph] -> ACC_Function/13(VVMC_MeterIndSpeedForCalcu_kph)
  SPD2ACC/8(VVMC_ISOJerkLimit_mps3) -> [VVMC_ISOJerkLimit_mps3]
  SPD2ACC/4(VVMC_SPD2ACCAct_flg) -> [VVMC_SPD2ACCAct_flg]
  Cast To Single21/1 -> VMC_FCM1/4(VINP_LKATOIFault_flg)  "VINP_LKATOIFault_flg"
  ACC_Function/2(VVMC_ACCPedalOvrd_flg) -> [VVMC_ACCPedalOvrd_flg]
  MSA function/1(VVMC_MSACtrlSta_enum) -> [VVMC_MSACtrlSta_enum]
  [VVMC_FeatArbitrFinal_enum] -> MSA function/8(VVMC_FeatArbitrFinal_enum)
  [VVMC_LongAcc_Gps] -> MSA function/6(VVMC_LongAcc_Gps)
  [VTQD_SWC1ResUpSta_flg] -> CruiseControlFunction/5(VTQD_SWC1ResUpSta_flg)  "VTQD_SWC1ResUpSta_flg"
  [VTQD_DriverWhlTqDem_Nm] -> CruiseControlFunction/2(VTQD_DriverWhlTqDem_Nm)  "VTQD_DriverWhlTqDem_Nm"
  [VINP_ADASAEBReq_enum] -> Cast To Single22/1
  Switch2/1 -> SpeedArbitration/11(VDSC_DISCTargetSpd_kph)  "VDSC_DISCTargetSpd_kph"
  [VVMC_FeatSetSpdForCalcu_kph] -> MSA function/7(VVMC_FeatSetSpdForCalcu_kph)
  [VVMC_CCSpdWar_flg] -> Logical Operator/1
  [VTQD_ExternalTqAllow_flg] -> CruiseControlFunction/1(VTQD_ExternalTqAllow_flg)  "VTQD_ExternalTqAllow_flg"
  Cast To Single19/1 -> VMC_FCM1/2(VINP_ADASLKASta_enum)  "VINP_ADASLKASta_enum"
  [VTQD_LowIdleAccPedal_flg] -> CruiseControlFunction/3(VTQD_LowIdleAccPedal_flg)  "VTQD_LowIdleAccPedal_flg"
  PreConditionCheck/3(VVMC_VMCCCCtrlAvail_flg) -> [VVMC_VMCCCCtrlAvail_flg]
  SPD2ACC/7(VVMC_ISODecLimit_mps2) -> [VVMC_ISODecLimit_mps2]
  [VVMC_JerkPCT_pct] -> SPD2ACC/5(VVMC_JerkPCT_pct)
  [VVMC_ACCCtrlAvail_flg] -> PreConditionCheck/10(VVMC_ACCCtrlAvail_flg)  "VVMC_ACCCtrlAvail_flg"
  [VVMC_VMCAEBCtrlAvail_flg] -> SpeedArbitration/4(VVMC_VMCAEBCtrlAvail_flg)
  MSA function/2(VVMC_MSAWhlTqReq_Nm) -> [VVMC_MSAWhlTqReq_Nm]
  [VTQD_SWC2CANCELSta_flg] -> MSA function/4(VTQD_SWC2CANCELSta_flg)  "VTQD_SWC2CANCELSta_flg"
  [VDSC_DISCTurn_flg] -> Switch5/3
  [VVMC_CCCtrlSta_enum] -> SpeedArbitration/9(VVMC_CCCtrlSta_enum)  "VVMC_CCCtrlSta_enum"
  SPD2ACC/5(VVMC_AccCalcuPID_mps2) -> [VVMC_AccCalcuPID_mps2]
  CruiseControlFunction/5(VVMC_CCPedalOvrd_flg) -> [VVMC_CCPedalOvrd_flg]
  [VVMC_FeatArbitrFinal_enum] -> ACC_Function/9(VVMC_FeatArbitrFinal_enum)
  FeatureSetSpeed/2(VVMC_FeatSetSpdForCalcu_kph) -> [VVMC_FeatSetSpdForCalcu_kph]
  [VVMC_VMCACCCtrlAvail_flg] -> SpeedArbitration/3(VVMC_VMCACCCtrlAvail_flg)
  SPD2ACC/6(VVMC_ISOAccLimit_mps2) -> [VVMC_ISOAccLimit_mps2]
  [VVMC_APSSpeedCMD_kph] -> VVMC_APSSpeedCMD_kph/1
  [VVMC_ACCCtrlAvail_flg] -> VVMC_ACCCtrlAvail_flg/1
  [VVMC_FeatSetSpdFinal_raw32] -> VVMC_FeatSetSpdFinal_raw32/1
  [VVMC_APSActive_flg] -> VVMC_APSActive_flg/1
  [VVMC_ADASActive_flg] -> VVMC_ADASActive_flg/1
  [VVMC_APSCtrlAvail_flg] -> VVMC_APSCtrlAvail_flg/1
  [VVMC_AEBVehHoldReq_flg] -> VVMC_AEBVehHoldReq_flg/1
  [VVMC_APSShiftPosnReq_enum] -> VVMC_APSShiftPosnReq_enum/1
  task_time_s/1 -> [task_time_s]  "task_time_s"
  VINP_DriverSeatBeltCmd_flg/1 -> [VINP_DriverSeatBeltCmd_flg]
  VTQD_ExternalTqAllow_flg/1 -> [VTQD_ExternalTqAllow_flg]
  VTQD_GearActualPosn_enum/1 -> [VTQD_GearActualPosn_enum]
  VTQD_ExtShftAllow_flg/1 -> [VTQD_ExtShftAllow_flg]
  VTQD_LowIdleAccPedal_flg/1 -> [VTQD_LowIdleAccPedal_flg]
  VTQD_CoordWhlTqDemRr_Nm/1 -> [VTQD_CoordWhlTqDemRr_Nm]
  VTQD_CoordWhlTqDemFr_Nm/1 -> [VTQD_CoordWhlTqDemFr_Nm]
  VTQD_DriverWhlTqDem_Nm/1 -> [VTQD_DriverWhlTqDem_Nm]
  VDSC_DISCTargetSpd_kph/1 -> [VDSC_DISCTargetSpd_kph]
  VDSC_DISCSta_enum/1 -> [VDSC_DISCSta_enum]
  VDSC_DISCTurn_flg/1 -> [VDSC_DISCTurn_flg]
  VBCM_DrDoorSW_flg/1 -> [VBCM_DrDoorSW_flg]
  VINP_APSSpeedCMD_kph/1 -> [VINP_APSSpeedCMD_kph]
  APP_SpdLimit/1 -> [APP_SpdLimit]
  APP_SpdLimit_flg/1 -> [APP_SpdLimit_flg]
  VINP_ADASAEBSta_enum/1 -> [VINP_ADASAEBSta_enum]
  VINP_LongAccel_Gps/1 -> [VINP_LongAccel_Gps]
  VTQD_SetSpd_kph/1 -> [VTQD_SetSpd_kph]
  VINP_LRRawWhlSpeedV_flg/1 -> [VINP_LRRawWhlSpeedV_flg]
  VTQD_SpdCtrlMode_enum/1 -> [VTQD_SpdCtrlMode_enum]
  VINP_LKAStrToqReq_Nm/1 -> [VINP_LKAStrToqReq_Nm]
  VINP_ACCRequiredAccel_mps2/1 -> [VINP_ACCRequiredAccel_mps2]
  VINP_ADASACCSta_enum/1 -> [VINP_ADASACCSta_enum]
  VINP_LatAccel_Gps/1 -> [VINP_LatAccel_Gps]
  VINP_LRRawWhlSpeed_kph/1 -> [VINP_LRRawWhlSpeed_kph]
  VTQD_SWC2ResUpSta_flg/1 -> [VTQD_SWC2ResUpSta_flg]
  VINP_ACCAvail_flg/1 -> [VINP_ACCAvail_flg]
  VINP_RRRawWhlSpeed_kph/1 -> [VINP_RRRawWhlSpeed_kph]
  VINP_LFRawWhlSpeedV_flg/1 -> [VINP_LFRawWhlSpeedV_flg]
  VTQD_SWC2CANCELSta_flg/1 -> [VTQD_SWC2CANCELSta_flg]
  VINP_ESCOFFStatus_enum/1 -> [VINP_ESCOFFStatus_enum]
  VINP_TimeGapLevel_enum/1 -> [VINP_TimeGapLevel_enum]
  VINP_AEBAvail_flg/1 -> [VINP_AEBAvail_flg]
  VINP_MeterIndVehSpeed_kph/1 -> [VINP_MeterIndVehSpeed_kph]
  VINP_AEBVehHoldReq_flg/1 -> [VINP_AEBVehHoldReq_flg]
  VINP_LKATOIFault_flg/1 -> [VINP_LKATOIFault_flg]
  VINP_LKATOIAct_enum/1 -> [VINP_LKATOIAct_enum]
  VINP_ACCObjRelSpd_mps/1 -> [VINP_ACCObjRelSpd_mps]
  VINP_ACCObjDist_m/1 -> [VINP_ACCObjDist_m]
  VINP_ACCVehHoldReq_flg/1 -> [VINP_ACCVehHoldReq_flg]
  VINP_BrkSwSta_flg/1 -> [VINP_BrkSwSta_flg]
  VINP_BrakeSWGPIO_flg/1 -> [VINP_BrakeSWGPIO_flg]
  VINP_RFRawWhlSpeed_kph/1 -> [VINP_RFRawWhlSpeed_kph]
  VINP_VehSpeed_kph/1 -> [VINP_VehSpeed_kph]
  VINP_EPBSta_enum/1 -> [VINP_EPBSta_enum]
  VINP_RRRawWhlSpeedV_flg/1 -> [VINP_RRRawWhlSpeedV_flg]
  VINP_LFRawWhlSpeed_kph/1 -> [VINP_LFRawWhlSpeed_kph]
  VINP_LatAccelV_flg/1 -> [VINP_LatAccelV_flg]
  VINP_GRADE_Deg/1 -> [VINP_GRADE_Deg]
  VINP_ADASDBSReq_enum/1 -> [VINP_ADASDBSReq_enum]
  VINP_RFRawWhlSpeedV_flg/1 -> [VINP_RFRawWhlSpeedV_flg]
  VTQD_SWC2SetdownSta_flg/1 -> [VTQD_SWC2SetdownSta_flg]
  VINP_ADASLKASta_enum/1 -> [VINP_ADASLKASta_enum]
  VTQD_SpdCtrlSta_flg/1 -> [VTQD_SpdCtrlSta_flg]
  VINP_ADASAEBReq_enum/1 -> [VINP_ADASAEBReq_enum]
  VINP_ADASFaultSta_flg/1 -> [VINP_ADASFaultSta_flg]
  [task_time_s] -> Long Acceleration Calculation/4(task_time_s)
  [VINP_RearAxlTrqReqBrk_Nm] -> ACC_Function/22(VINP_RearAxlTrqReqBrk_Nm)  "VINP_RearAxlTrqReqBrk_Nm"
  [VINP_FrntAxlTrqReqBrk_Nm] -> ACC_Function/21(VINP_FrntAxlTrqReqBrk_Nm)  "VINP_FrntAxlTrqReqBrk_Nm"
  [VTQD_SWC2ResUpSta_flg] -> ACC_Function/20(VTQD_SWC2ResUpSta_flg)
  VINP_FrntAxlTrqReqBrk_Nm/1 -> [VINP_FrntAxlTrqReqBrk_Nm]
  VINP_RearAxlTrqReqBrk_Nm/1 -> [VINP_RearAxlTrqReqBrk_Nm]
  ACC_Function/6(VVMC_ADASNegReq_flg) -> [VVMC_ADASNegReq_flg]
  [VTQD_GearActualPosn_enum] -> CruiseControlFunction/15(VTQD_GearActualPosn_enum)
  [Trigger_10ms_2] -> SafetyControl/Trigger
  VTQR_RrTMTqReq_Nm/1 -> [VTQR_RrTMTqReq_Nm]
  [VTQR_RrTMTqReq_Nm] -> Unit Delay/1
  Unit Delay/1 -> ACC_Function/23(VTQR_RrTMTqReq_Nm)
  [VVMC_LongAcc_Gps] -> SPD2ACC/11(VVMC_LongAcc_Gps)
  ACC_Function/7(VVMC_AccPedalOvrdDISC_flg) -> [VVMC_AccPedalOvrdDISC_flg]
  [Trigger_10ms_1] -> SpeedCalculation/Trigger
  VINP_ACCJerkUpperLimit_mps3/1 -> [VINP_ACCJerkUpperLimit_mps3]
  VINP_ACCComfortBandUpper_mps2/1 -> [VINP_ACCComfortBandUpper_mps2]
  VINP_ACCJerkLowerLimit_mps3/1 -> [VINP_ACCJerkLowerLimit_mps3]
  VINP_ACCComfortBandLower_mps2/1 -> [VINP_ACCComfortBandLower_mps2]
  VINP_ADASVehSpdLim_raw32/1 -> [VINP_ADASVehSpdLim_raw32]
  VINP_ADASShftPosnReqA_flg/1 -> [VINP_ADASShftPosnReqA_flg]
  VINP_ADASShftPosnReq_enum/1 -> [VINP_ADASShftPosnReq_enum]
  VINP_ADASForceIdle_flg/1 -> [VINP_ADASForceIdle_flg]
  VINP_HazardWarningReq_flg/1 -> [VINP_HazardWarningReq_flg]
  VINP_RightTurnLightReq_flg/1 -> [VINP_RightTurnLightReq_flg]
  VINP_LeftTurnLightReq_flg/1 -> [VINP_LeftTurnLightReq_flg]
  VINP_ADASFCWSta_enum/1 -> [VINP_ADASFCWSta_enum]
  VINP_ADASLDWSta_enum/1 -> [VINP_ADASLDWSta_enum]
  VINP_ADASFltWrnReq_flg/1 -> [VINP_ADASFltWrnReq_flg]
  VINP_ACCObjDstLvl_enum/1 -> [VINP_ACCObjDstLvl_enum]
  VINP_ForceLowBeam_enum/1 -> [VINP_ForceLowBeam_enum]
  VINP_ACCTakeoverReq_flg/1 -> [VINP_ACCTakeoverReq_flg]
  VINP_ADASWarningMsg_enum/1 -> [VINP_ADASWarningMsg_enum]
  VINP_ADASCAMSpdLim_enum/1 -> [VINP_ADASCAMSpdLim_enum]
  VINP_TargetType_enum/1 -> [VINP_TargetType_enum]
  VINP_ADASSLIFSpdLim_enum/1 -> [VINP_ADASSLIFSpdLim_enum]
  VINP_LKAHODDisplayWarning_flg/1 -> [VINP_LKAHODDisplayWarning_flg]
  VINP_LKAHODSoundWarning_flg/1 -> [VINP_LKAHODSoundWarning_flg]
  VINP_ADASLFCSta_enum/1 -> [VINP_ADASLFCSta_enum]
  VINP_ADASLaneModeL_enum/1 -> [VINP_ADASLaneModeL_enum]
  VINP_ADASLaneModeR_enum/1 -> [VINP_ADASLaneModeR_enum]
  VINP_ADASSLIFSta_enum/1 -> [VINP_ADASSLIFSta_enum]
  VINP_ADASISASta_enum/1 -> [VINP_ADASISASta_enum]
  VINP_ADASLDWMute_flg/1 -> [VINP_ADASLDWMute_flg]
  VINP_ADASFCWMute_flg/1 -> [VINP_ADASFCWMute_flg]
  VINP_ADASLFCHandsOffWarning_enum/1 -> [VINP_ADASLFCHandsOffWarning_enum]
  VINP_LVDADisabled_flg/1 -> [VINP_LVDADisabled_flg]
  VINP_LVDAMuteSta_enum/1 -> [VINP_LVDAMuteSta_enum]
  VINP_LVDAFailinfo_flg/1 -> [VINP_LVDAFailinfo_flg]
  VINP_LVDAWarning_flg/1 -> [VINP_LVDAWarning_flg]
  VINP_LVDAACCStatusInformation_flg/1 -> [VINP_LVDAACCStatusInformation_flg]
  VINP_ADASLFCWarnSound_enum/1 -> [VINP_ADASLFCWarnSound_enum]
  VINP_FCMACCmode_enum/1 -> [VINP_FCMACCmode_enum]
  VINP_ADASLanetypeR_enum/1 -> [VINP_ADASLanetypeR_enum]
  VINP_ADASLanetypeL_enum/1 -> [VINP_ADASLanetypeL_enum]
  VINP_ADASLanecurveL_raw32/1 -> [VINP_ADASLanecurveL_raw32]
  VINP_ADASLanecurveR_raw32/1 -> [VINP_ADASLanecurveR_raw32]
  [VINP_ACCObjDist_m] -> Cast To Single4/1
  [VINP_ACCObjRelSpd_mps] -> Cast To Single3/1
  [VINP_TimeGapLevel_enum] -> Cast To Single1/1
  Cast To Single1/1 -> VMC_FCM1/14(VINP_TimeGapLevel_enum)  "VINP_TimeGapLevel_enum"
  Cast To Single3/1 -> VMC_FCM1/13(VINP_ACCObjRelSpd_mps)  "VINP_ACCObjRelSpd_mps"
  Cast To Single4/1 -> VMC_FCM1/12(VINP_ACCObjDist_m)  "VINP_ACCObjDist_m"
  [VINP_ACCJerkUpperLimit_mps3] -> Cast To Single5/1
  Cast To Single5/1 -> VMC_FCM1/15(VINP_ACCJerkUpperLimit_mps3)  "VINP_ACCJerkUpperLimit_mps3"
  [VINP_ACCComfortBandUpper_mps2] -> Cast To Single6/1
  Cast To Single6/1 -> VMC_FCM1/16(VINP_ACCComfortBandUpper_mps2)  "VINP_ACCComfortBandUpper_mps2"
  [VINP_ACCJerkLowerLimit_mps3] -> Cast To Single8/1
  Cast To Single8/1 -> VMC_FCM1/17(VINP_ACCJerkLowerLimit_mps3)  "VINP_ACCJerkLowerLimit_mps3"
  [VINP_ACCComfortBandLower_mps2] -> Cast To Single9/1
  Cast To Single9/1 -> VMC_FCM1/18(VINP_ACCComfortBandLower_mps2)  "VINP_ACCComfortBandLower_mps2"
  [VINP_ADASVehSpdLim_raw32] -> Cast To Single10/1
  Cast To Single10/1 -> VMC_FCM1/19(VINP_ADASVehSpdLim_raw32)  "VINP_ADASVehSpdLim_raw32"
  [VINP_ADASShftPosnReqA_flg] -> Cast To Single11/1
  Cast To Single11/1 -> VMC_FCM1/20(VINP_ADASShftPosnReqA_flg)  "VINP_ADASShftPosnReqA_flg"
  [VINP_ADASShftPosnReq_enum] -> Cast To Single12/1
  Cast To Single12/1 -> VMC_FCM1/21(VINP_ADASShftPosnReq_enum)  "VINP_ADASShftPosnReq_enum"
  [VINP_ADASForceIdle_flg] -> Cast To Single13/1
  Cast To Single13/1 -> VMC_FCM1/22(VINP_ADASForceIdle_flg)  "VINP_ADASForceIdle_flg"
  [VINP_HazardWarningReq_flg] -> Cast To Single14/1
  Cast To Single14/1 -> VMC_FCM1/23(VINP_HazardWarningReq_flg)  "VINP_HazardWarningReq_flg"
  [VINP_RightTurnLightReq_flg] -> Cast To Single15/1
  Cast To Single15/1 -> VMC_FCM1/24(VINP_RightTurnLightReq_flg)  "VINP_RightTurnLightReq_flg"
  [VINP_LeftTurnLightReq_flg] -> Cast To Single16/1
  Cast To Single16/1 -> VMC_FCM1/25(VINP_LeftTurnLightReq_flg)  "VINP_LeftTurnLightReq_flg"
  Cast To Single17/1 -> VMC_FCM1/26(VINP_ADASFCWSta_enum)  "VINP_ADASFCWSta_enum"
  [VINP_ADASFCWSta_enum] -> Cast To Single17/1
  [VINP_ADASLDWSta_enum] -> Cast To Single26/1
  Cast To Single26/1 -> VMC_FCM1/27(VINP_ADASLDWSta_enum)  "VINP_ADASLDWSta_enum"
  [VINP_ADASFltWrnReq_flg] -> Cast To Single27/1
  Cast To Single27/1 -> VMC_FCM1/28(VINP_ADASFltWrnReq_flg)  "VINP_ADASFltWrnReq_flg"
  Cast To Single29/1 -> VMC_FCM1/29(VINP_ACCObjDstLvl_enum)  "VINP_ACCObjDstLvl_enum"
  [VINP_ACCObjDstLvl_enum] -> Cast To Single29/1
  [VINP_ForceLowBeam_enum] -> Cast To Single30/1
  Cast To Single30/1 -> VMC_FCM1/30(VINP_ForceLowBeam_enum)  "VINP_ForceLowBeam_enum"
  [VINP_ACCTakeoverReq_flg] -> Cast To Single37/1
  Cast To Single37/1 -> VMC_FCM1/31(VINP_ACCTakeoverReq_flg)  "VINP_ACCTakeoverReq_flg"
  [VINP_ADASWarningMsg_enum] -> Cast To Single36/1
  Cast To Single36/1 -> VMC_FCM1/32(VINP_ADASWarningMsg_enum)  "VINP_ADASWarningMsg_enum"
  [VINP_ADASCAMSpdLim_enum] -> Cast To Single38/1
  Cast To Single38/1 -> VMC_FCM1/33(VINP_ADASCAMSpdLim_enum)  "VINP_ADASCAMSpdLim_enum"
  [VINP_TargetType_enum] -> Cast To Single39/1
  Cast To Single39/1 -> VMC_FCM1/34(VINP_TargetType_enum)  "VINP_TargetType_enum"
  [VINP_ADASSLIFSpdLim_enum] -> Cast To Single40/1
  Cast To Single40/1 -> VMC_FCM1/35(VINP_ADASSLIFSpdLim_enum)  "VINP_ADASSLIFSpdLim_enum"
  [VINP_LKAHODDisplayWarning_flg] -> Cast To Single41/1
  Cast To Single41/1 -> VMC_FCM1/36(VINP_LKAHODDisplayWarning_flg)  "VINP_LKAHODDisplayWarning_flg"
  [VINP_LKAHODSoundWarning_flg] -> Cast To Single42/1
  Cast To Single42/1 -> VMC_FCM1/37(VINP_LKAHODSoundWarning_flg)  "VINP_LKAHODSoundWarning_flg"
  [VINP_ADASLFCSta_enum] -> Cast To Single43/1
  Cast To Single43/1 -> VMC_FCM1/38(VINP_ADASLFCSta_enum)  "VINP_ADASLFCSta_enum"
  [VINP_ADASLaneModeL_enum] -> Cast To Single44/1
  Cast To Single44/1 -> VMC_FCM1/39(VINP_ADASLaneModeL_enum)  "VINP_ADASLaneModeL_enum"
  [VINP_ADASLaneModeR_enum] -> Cast To Single45/1
  Cast To Single45/1 -> VMC_FCM1/40(VINP_ADASLaneModeR_enum)  "VINP_ADASLaneModeR_enum"
  [VINP_ADASSLIFSta_enum] -> Cast To Single46/1
  Cast To Single46/1 -> VMC_FCM1/41(VINP_ADASSLIFSta_enum)  "VINP_ADASSLIFSta_enum"
  [VINP_ADASISASta_enum] -> Cast To Single47/1
  Cast To Single47/1 -> VMC_FCM1/42(VINP_ADASISASta_enum)  "VINP_ADASISASta_enum"
  [VINP_ADASLDWMute_flg] -> Cast To Single48/1
  Cast To Single48/1 -> VMC_FCM1/43(VINP_ADASLDWMute_flg)  "VINP_ADASLDWMute_flg"
  [VINP_ADASFCWMute_flg] -> Cast To Single49/1
  Cast To Single49/1 -> VMC_FCM1/44(VINP_ADASFCWMute_flg)  "VINP_ADASFCWMute_flg"
  [VINP_ADASLFCHandsOffWarning_enum] -> Cast To Single50/1
  Cast To Single50/1 -> VMC_FCM1/45(VINP_ADASLFCHandsOffWarning_enum)  "VINP_ADASLFCHandsOffWarning_enum"
  [VINP_LVDADisabled_flg] -> Cast To Single51/1
  Cast To Single51/1 -> VMC_FCM1/46(VINP_LVDADisabled_flg)  "VINP_LVDADisabled_flg"
  [VINP_LVDAMuteSta_enum] -> Cast To Single52/1
  Cast To Single52/1 -> VMC_FCM1/47(VINP_LVDAMuteSta_enum)  "VINP_LVDAMuteSta_enum"
  [VINP_LVDAFailinfo_flg] -> Cast To Single53/1
  Cast To Single53/1 -> VMC_FCM1/48(VINP_LVDAFailinfo_flg)  "VINP_LVDAFailinfo_flg"
  [VINP_LVDAWarning_flg] -> Cast To Single54/1
  Cast To Single54/1 -> VMC_FCM1/49(VINP_LVDAWarning_flg)  "VINP_LVDAWarning_flg"
  [VINP_LVDAACCStatusInformation_flg] -> Cast To Single55/1
  Cast To Single55/1 -> VMC_FCM1/50(VINP_LVDAACCStatusInformation_flg)  "VINP_LVDAACCStatusInformation_flg"
  [VINP_ADASLFCWarnSound_enum] -> Cast To Single56/1
  Cast To Single56/1 -> VMC_FCM1/51(VINP_ADASLFCWarnSound_enum)  "VINP_ADASLFCWarnSound_enum"
  [VINP_FCMACCmode_enum] -> Cast To Single57/1
  Cast To Single57/1 -> VMC_FCM1/52(VINP_FCMACCmode_enum)  "VINP_FCMACCmode_enum"
  [VINP_ADASLanetypeR_enum] -> Cast To Single58/1
  Cast To Single58/1 -> VMC_FCM1/53(VINP_ADASLanetypeR_enum)  "VINP_ADASLanetypeR_enum"
  [VINP_ADASLanetypeL_enum] -> Cast To Single59/1
  Cast To Single59/1 -> VMC_FCM1/54(VINP_ADASLanetypeL_enum)  "VINP_ADASLanetypeL_enum"
  [VINP_ADASLanecurveL_raw32] -> Cast To Single60/1
  Cast To Single60/1 -> VMC_FCM1/55(VINP_ADASLanecurveL_raw32)  "VINP_ADASLanecurveL_raw32"
  [VINP_ADASLanecurveR_raw32] -> Cast To Single61/1
  Cast To Single61/1 -> VMC_FCM1/56(VINP_ADASLanecurveR_raw32)  "VINP_ADASLanecurveR_raw32"
  VMC_FCM1/1(VVMC_LateralCtrl_flg) -> [VVMC_LateralCtrl_flg]
  VMC_FCM1/2(VVMC_ADASLKASta_enum) -> [VVMC_ADASLKASta_enum]  "VVMC_ADASLKASta_enum"
  VMC_FCM1/3(VVMC_LKAStrToqReq_Nm) -> [VVMC_LKAStrToqReq_Nm]  "VVMC_LKAStrToqReq_Nm"
  VMC_FCM1/4(VVMC_LKATOIFault_flg) -> [VVMC_LKATOIFault_flg]  "VVMC_LKATOIFault_flg"
  VMC_FCM1/5(VVMC_LKATOIAct_enum) -> [VVMC_LKATOIAct_enum]  "VVMC_LKATOIAct_enum"
  VMC_FCM1/6(VVMC_ADASAEBReq_enum) -> [VVMC_ADASAEBReq_enum]  "VVMC_ADASAEBReq_enum"
  VMC_FCM1/7(VVMC_ADASFaultSta_flg) -> [VVMC_ADASFaultSta_flg]  "VVMC_ADASFaultSta_flg"
  VMC_FCM1/8(VVMC_AEBVehHoldReq_flg) -> [VVMC_AEBVehHoldReq_flg]  "VVMC_AEBVehHoldReq_flg"
  VMC_FCM1/10(VVMC_ADASDBSReq_enum) -> [VVMC_ADASDBSReq_enum]  "VVMC_ADASDBSReq_enum"
  VMC_FCM1/12(VVMC_ACCObjDist_m) -> [VVMC_ACCObjDist_m]  "VVMC_ACCObjDist_m"
  VMC_FCM1/13(VVMC_ACCObjRelSpd_mps) -> [VVMC_ACCObjRelSpd_mps]  "VVMC_ACCObjRelSpd_mps"
  VMC_FCM1/14(VVMC_TimeGapLevel_enum) -> [VVMC_TimeGapLevel_enum]  "VVMC_TimeGapLevel_enum"
  VMC_FCM1/15(VVMC_ACCJerkUpperLimit_mps3) -> [VVMC_ACCJerkUpperLimit_mps3]  "VVMC_ACCJerkUpperLimit_mps3"
  VMC_FCM1/16(VVMC_ACCComfortBandUpper_mps2) -> [VVMC_ACCComfortBandUpper_mps2]  "VVMC_ACCComfortBandUpper_mps2"
  VMC_FCM1/17(VVMC_ACCJerkLowerLimit_mps3) -> [VVMC_ACCJerkLowerLimit_mps3]  "VVMC_ACCJerkLowerLimit_mps3"
  VMC_FCM1/18(VVMC_ACCComfortBandLower_mps2) -> [VVMC_ACCComfortBandLower_mps2]  "VVMC_ACCComfortBandLower_mps2"
  VMC_FCM1/19(VVMC_ADASVehSpdLim_raw32) -> [VVMC_ADASVehSpdLim_raw32]  "VVMC_ADASVehSpdLim_raw32"
  VMC_FCM1/20(VVMC_ADASShftPosnReqA_flg) -> [VVMC_ADASShftPosnReqA_flg]  "VVMC_ADASShftPosnReqA_flg"
  VMC_FCM1/21(VVMC_ADASShftPosnReq_enum) -> [VVMC_ADASShftPosnReq_enum]  "VVMC_ADASShftPosnReq_enum"
  VMC_FCM1/22(VVMC_ADASForceIdle_flg) -> [VVMC_ADASForceIdle_flg]  "VVMC_ADASForceIdle_flg"
  VMC_FCM1/23(VVMC_HazardWarningReq_flg) -> [VVMC_HazardWarningReq_flg]  "VVMC_HazardWarningReq_flg"
  VMC_FCM1/24(VVMC_RightTurnLightReq_flg) -> [VVMC_RightTurnLightReq_flg]  "VVMC_RightTurnLightReq_flg"
  VMC_FCM1/25(VVMC_LeftTurnLightReq_flg) -> [VVMC_LeftTurnLightReq_flg]  "VVMC_LeftTurnLightReq_flg"
  VMC_FCM1/26(VVMC_ADASFCWSta_enum) -> [VVMC_ADASFCWSta_enum]  "VVMC_ADASFCWSta_enum"
  VMC_FCM1/27(VVMC_ADASLDWSta_enum) -> [VVMC_ADASLDWSta_enum]  "VVMC_ADASLDWSta_enum"
  VMC_FCM1/28(VVMC_ADASFltWrnReq_flg) -> [VVMC_ADASFltWrnReq_flg]  "VVMC_ADASFltWrnReq_flg"
  VMC_FCM1/29(VVMC_ACCObjDstLvl_enum) -> [VVMC_ACCObjDstLvl_enum]  "VVMC_ACCObjDstLvl_enum"
  VMC_FCM1/30(VVMC_ForceLowBeam_enum) -> [VVMC_ForceLowBeam_enum]  "VVMC_ForceLowBeam_enum"
  VMC_FCM1/31(VVMC_ACCTakeoverReq_flg) -> [VVMC_ACCTakeoverReq_flg]  "VVMC_ACCTakeoverReq_flg"
  VMC_FCM1/32(VVMC_ADASWarningMsg_enum) -> [VVMC_ADASWarningMsg_enum]  "VVMC_ADASWarningMsg_enum"
  VMC_FCM1/33(VVMC_ADASCAMSpdLim_enum) -> [VVMC_ADASCAMSpdLim_enum]  "VVMC_ADASCAMSpdLim_enum"
  VMC_FCM1/34(VVMC_TargetType_enum) -> [VVMC_TargetType_enum]  "VVMC_TargetType_enum"
  VMC_FCM1/35(VVMC_ADASSLIFSpdLim_enum) -> [VVMC_ADASSLIFSpdLim_enum]  "VVMC_ADASSLIFSpdLim_enum"
  VMC_FCM1/36(VVMC_LKAHODDisplayWarning_flg) -> [VVMC_LKAHODDisplayWarning_flg]  "VVMC_LKAHODDisplayWarning_flg"
  VMC_FCM1/37(VVMC_LKAHODSoundWarning_flg) -> [VVMC_LKAHODSoundWarning_flg]  "VVMC_LKAHODSoundWarning_flg"
  VMC_FCM1/38(VVMC_ADASLFCSta_enum) -> [VVMC_ADASLFCSta_enum]  "VVMC_ADASLFCSta_enum"
  VMC_FCM1/39(VVMC_ADASLaneModeL_enum) -> [VVMC_ADASLaneModeL_enum]  "VVMC_ADASLaneModeL_enum"
  VMC_FCM1/40(VVMC_ADASLaneModeR_enum) -> [VVMC_ADASLaneModeR_enum]  "VVMC_ADASLaneModeR_enum"
  VMC_FCM1/41(VVMC_ADASSLIFSta_enum) -> [VVMC_ADASSLIFSta_enum]  "VVMC_ADASSLIFSta_enum"
  VMC_FCM1/42(VVMC_ADASISASta_enum) -> [VVMC_ADASISASta_enum]  "VVMC_ADASISASta_enum"
  VMC_FCM1/43(VVMC_ADASLDWMute_flg) -> [VVMC_ADASLDWMute_flg]  "VVMC_ADASLDWMute_flg"
  VMC_FCM1/44(VVMC_ADASFCWMute_flg) -> [VVMC_ADASFCWMute_flg]  "VVMC_ADASFCWMute_flg"
  VMC_FCM1/45(VVMC_ADASLFCHandsOffWarning_enum) -> [VVMC_ADASLFCHandsOffWarning_enum]  "VVMC_ADASLFCHandsOffWarning_enum"
  VMC_FCM1/46(VVMC_LVDADisabled_flg) -> [VVMC_LVDADisabled_flg]  "VVMC_LVDADisabled_flg"
  VMC_FCM1/47(VVMC_LVDAMuteSta_enum) -> [VVMC_LVDAMuteSta_enum]  "VVMC_LVDAMuteSta_enum"
  VMC_FCM1/48(VVMC_LVDAFailinfo_flg) -> [VVMC_LVDAFailinfo_flg]  "VVMC_LVDAFailinfo_flg"
  VMC_FCM1/49(VVMC_LVDAWarning_flg) -> [VVMC_LVDAWarning_flg]  "VVMC_LVDAWarning_flg"
  VMC_FCM1/50(VVMC_LVDAACCStatusInformation_flg) -> [VVMC_LVDAACCStatusInformation_flg]  "VVMC_LVDAACCStatusInformation_flg"
  VMC_FCM1/51(VVMC_ADASLFCWarnSound_enum) -> [VVMC_ADASLFCWarnSound_enum]  "VVMC_ADASLFCWarnSound_enum"
  VMC_FCM1/52(VVMC_FCMACCmode_enum) -> [VVMC_FCMACCmode_enum]  "VVMC_FCMACCmode_enum"
  VMC_FCM1/53(VVMC_ADASLanetypeR_enum) -> [VVMC_ADASLanetypeR_enum]  "VVMC_ADASLanetypeR_enum"
  VMC_FCM1/54(VVMC_ADASLanetypeL_enum) -> [VVMC_ADASLanetypeL_enum]  "VVMC_ADASLanetypeL_enum"
  VMC_FCM1/55(VVMC_ADASLanecurveL_raw32) -> [VVMC_ADASLanecurveL_raw32]  "VVMC_ADASLanecurveL_raw32"
  VMC_FCM1/56(VVMC_ADASLanecurveR_raw32) -> [VVMC_ADASLanecurveR_raw32]  "VVMC_ADASLanecurveR_raw32"
  [VINP_ADASAEBSta_enum] -> Cast To Single62/1
  Cast To Single62/1 -> VMC_FCM1/57(VINP_ADASAEBSta_enum)  "VINP_ADASAEBSta_enum"
  VMC_FCM1/57(VVMC_ADASAEBSta_enum) -> [VVMC_ADASAEBSta_enum]  "VVMC_ADASAEBSta_enum"
  Function-Call Split/2 -> [Trigger_10ms_2]
  Scheduler/1(Trigger_10ms_1()) -> Function-Call Split/1
  Function-Call Split/1 -> [Trigger_10ms_1]
  [VVMC_ACCVehHoldReqRaw_flg] -> ACC_Function/24(VVMC_ACCVehHoldReqRaw_flg)
  VMC_FCM1/58(VVMC_FCMLDWRequest_enum) -> [VVMC_FCMLDWRequest_enum]
  VMC_FCM1/59(VVMC_FCMLDWFault_flg) -> [VVMC_FCMLDWFault_flg]
  VINP_BrkPedalPos_pct/1 -> [VINP_BrkPedalPos_pct]
  [VVMC_ADASWhlTqReq_Nm] -> Unit Delay1/1
  Unit Delay1/1 -> SPD2ACC/12(VVMC_LastADASWhlTqReq_Nm)  "VVMC_LastADASWhlTqReq_Nm"
  [VTQD_RrEDUAvailBrkRgnTq_Nm] -> SPD2ACC/13(VTQD_RrEDUAvailBrkRgnTq_Nm)  "VTQD_RrEDUAvailBrkRgnTq_Nm"
  VTQD_RrEDUAvailBrkRgnTq_Nm/1 -> [VTQD_RrEDUAvailBrkRgnTq_Nm]
  SPD2ACC/9(VVMC_ActACCRequiredAccel_mps2) -> [VVMC_ActACCRequiredAccel_mps2]
  [VVMC_EstSlope_Deg] -> ACC_Function/25(VVMC_EstSlope_Deg)
  [VVMC_EstSlopeCal_Deg] -> Long Acceleration Calculation/5(VVMC_EstSlopeCal_Deg)
  [VVMC_FeatSetSpdForCalcu_kph] -> Long Acceleration Calculation/6(VVMC_FeatSetSpdForCalcu_kph)
  [VVMC_MeterIndSpeedForCalcu_kph] -> MSA function/11(VVMC_MeterIndSpeedForCalcu_kph)
  VDHP_ActAPSPosn_pct/1 -> [VDHP_ActAPSPosn_pct]
  [VTQD_LowIdleAccPedal_flg] -> MSA function/12(VTQD_LowIdleAccPedal_flg)  "VTQD_LowIdleAccPedal_flg"
  [VDHP_ActAPSPosn_pct] -> MSA function/13(VDHP_ActAPSPosn_pct)  "VDHP_ActAPSPosn_pct"
  [task_time_s] -> MSA function/14(task_time_s)  "task_time_s"
  VTQD_APSReq_enum/1 -> [VTQD_APSReq_enum]
  VTQD_APSDecReq_mps2/1 -> [VTQD_APSDecReq_mps2]
  VTQD_APSDecReqA_flg/1 -> [VTQD_APSDecReqA_flg]
  VTQD_APSStaSys_enum/1 -> [VTQD_APSStaSys_enum]
  VTQD_EquivAccPedalSWSta_flg/1 -> [VTQD_EquivAccPedalSWSta_flg]
  VTQD_AfterAvailableTqDemRr_Nm/1 -> [VTQD_AfterAvailableTqDemRr_Nm]
  VTQD_AfterAvailableTqDemFr_Nm/1 -> [VTQD_AfterAvailableTqDemFr_Nm]
  [VVMC_LongAccelCalcuByVehSpdRaw_gps] -> Long Acceleration Calculation/7(VVMC_LongAccelCalcuByVehSpdRaw_gps)
  [VINP_TargetType_enum] -> ACC_Function/26(VINP_TargetType_enum)
  [VVMC_SafetyCtrl_flg] -> ACC_Function/27(VVMC_SafetyCtrl_flg)
  ACC_Function/8(VVMC_RearTqRatio_rat) -> [VVMC_RearTqRatio_rat]
  [VINP_LongAccel_Gps] -> ACC_Function/28(VINP_LongAccel_Gps)  "VINP_LongAccel_Gps"
  [VVMC_FrRrSlipSpd_kph] -> ACC_Function/29(VVMC_FrRrSlipSpd_kph)
  [VVMC_CruzWhlTqReq_Nm] -> ACC_Function/30(VVMC_CruzWhlTqReq_Nm)
  [VVMC_CruzActive_flg] -> ACC_Function/31(VVMC_CruzActive_flg)
  [VVMC_MSAWhlTqReq_Nm] -> ACC_Function/32(VVMC_MSAWhlTqReq_Nm)
  [VVMC_MSAActive_flg] -> ACC_Function/33(VVMC_MSAActive_flg)
  [VVMC_VehicleSpeed_mph] -> VVMC_VehicleSpeed_mph/1
  [VVMC_VehicleSpeed_kph] -> VVMC_VehicleSpeed_kph/1
  [VVMC_MeterIndSpeed_raw32] -> VVMC_MeterIndSpeed_raw32/1
  [VVMC_MeterIndSpeedForCalcu_kph] -> VVMC_MeterIndSpeedForCalcu_kph/1
  [VVMC_VMCACCCtrlAvail_flg] -> VVMC_VMCACCCtrlAvail_flg/1
  [VVMC_VMCCCCtrlAvail_flg] -> VVMC_VMCCCCtrlAvail_flg/1
  [VVMC_VMCMSACtrlAvail_flg] -> VVMC_VMCMSACtrlAvail_flg/1
  [VVMC_VMCAEBCtrlAvail_flg] -> VVMC_VMCAEBCtrlAvail_flg/1
  [VVMC_JerkPCT_pct] -> VVMC_JerkPCT_pct/1
  [VVMC_LimitPCT_pct] -> VVMC_LimitPCT_pct/1
  [VVMC_FeatArbitrSta_enum] -> VVMC_FeatArbitrSta_enum/1  "VVMC_FeatArbitrSta_enum"
  [VVMC_FeatReqSpd_kph] -> VVMC_FeatReqSpd_kph/1
  [VVMC_LFWhlSpeedRollAve_kph] -> VVMC_LFWhlSpeedRollAve_kph/1  "VVMC_LFWhlSpeedRollAve_kph"
  [VVMC_RFWhlSpeedRollAve_kph] -> VVMC_RFWhlSpeedRollAve_kph/1  "VVMC_RFWhlSpeedRollAve_kph"
  [VVMC_RRWhlSpeedRollAve_kph] -> VVMC_RRWhlSpeedRollAve_kph/1  "VVMC_RRWhlSpeedRollAve_kph"
  [VVMC_LRWhlSpeedRollAve_kph] -> VVMC_LRWhlSpeedRollAve_kph/1  "VVMC_LRWhlSpeedRollAve_kph"
  [VVMC_LatAccCtrl_flg] -> VVMC_LatAccCtrl_flg/1
  [VVMC_RearWhlSlipRatioCtrl_flg] -> VVMC_RearWhlSlipRatioCtrl_flg/1
  [VVMC_FrontRearSlipRatioCtrl_flg] -> VVMC_FrontRearSlipRatioCtrl_flg/1
  [VVMC_SingleWhlSlipRatioCtrl_flg] -> VVMC_SingleWhlSlipRatioCtrl_flg/1
  [VVMC_SafetyCtrl_flg] -> VVMC_SafetyCtrl_flg/1
  [VVMC_ISOJerkLimit_mps3] -> VVMC_ISOJerkLimit_mps3/1
  [VVMC_SPD2ACCAct_flg] -> VVMC_SPD2ACCAct_flg/1
  [VVMC_ISOAccLimit_mps2] -> VVMC_ISOAccLimit_mps2/1
  [VVMC_AccCalcuPID_mps2] -> VVMC_AccCalcuPID_mps2/1
  [VVMC_ISODecLimit_mps2] -> VVMC_ISODecLimit_mps2/1
  [VVMC_DISCReqAcc_mps2] -> VVMC_DISCReqAcc_mps2/1  "VVMC_DISCReqAcc_mps2"
  [VVMC_ACCRequiredAccel_mps2] -> VVMC_ACCRequiredAccel_mps2/1
  [VVMC_ActACCRequiredAccel_mps2] -> VVMC_ActACCRequiredAccel_mps2/1
  [VVMC_FeatArbitrFinal_enum] -> VVMC_FeatArbitrFinal_enum/1
  [VVMC_LateralCtrl_flg] -> VVMC_LateralCtrl_flg/1
  [VVMC_ADASLKASta_enum] -> VVMC_ADASLKASta_enum/1
  [VVMC_LKATOIAct_enum] -> VVMC_LKATOIAct_enum/1
  [VVMC_LKAStrToqReq_Nm] -> VVMC_LKAStrToqReq_Nm/1
  [VVMC_LKATOIFault_flg] -> VVMC_LKATOIFault_flg/1
  [VVMC_ADASAEBSta_enum] -> VVMC_ADASAEBSta_enum/1
  [VVMC_ADASFaultSta_flg] -> VVMC_ADASFaultSta_flg/1
  [VVMC_ACCVehHoldReq_flg] -> VVMC_ACCVehHoldReq_flg/1  "VVMC_ACCVehHoldReq_flg"
  [VVMC_ADASDBSReq_enum] -> VVMC_ADASDBSReq_enum/1
  [VVMC_ADASACCSta_enum] -> VVMC_ADASACCSta_enum/1  "VVMC_ADASACCSta_enum"
  [VVMC_ACCObjRelSpd_mps] -> VVMC_ACCObjRelSpd_mps/1
  [VVMC_ACCObjDist_m] -> VVMC_ACCObjDist_m/1
  [VVMC_TimeGapLevel_enum] -> VVMC_TimeGapLevel_enum/1
  [VVMC_ACCJerkLowerLimit_mps3] -> VVMC_ACCJerkLowerLimit_mps3/1
  [VVMC_ACCComfortBandLower_mps2] -> VVMC_ACCComfortBandLower_mps2/1
  [VVMC_ACCJerkUpperLimit_mps3] -> VVMC_ACCJerkUpperLimit_mps3/1
  [VVMC_ACCComfortBandUpper_mps2] -> VVMC_ACCComfortBandUpper_mps2/1
  [VVMC_ADASVehSpdLim_raw32] -> VVMC_ADASVehSpdLim_raw32/1
  [VVMC_ADASShftPosnReqA_flg] -> VVMC_ADASShftPosnReqA_flg/1
  [VVMC_ADASShftPosnReq_enum] -> VVMC_ADASShftPosnReq_enum/1
  [VVMC_ADASForceIdle_flg] -> VVMC_ADASForceIdle_flg/1
  [VVMC_LeftTurnLightReq_flg] -> VVMC_LeftTurnLightReq_flg/1
  [VVMC_HazardWarningReq_flg] -> VVMC_HazardWarningReq_flg/1
  [VVMC_RightTurnLightReq_flg] -> VVMC_RightTurnLightReq_flg/1
  [VVMC_ADASFltWrnReq_flg] -> VVMC_ADASFltWrnReq_flg/1
  [VVMC_ADASFCWSta_enum] -> VVMC_ADASFCWSta_enum/1
  [VVMC_ADASLDWSta_enum] -> VVMC_ADASLDWSta_enum/1
  [VVMC_ACCTakeoverReq_flg] -> VVMC_ACCTakeoverReq_flg/1
  [VVMC_ForceLowBeam_enum] -> VVMC_ForceLowBeam_enum/1
  [VVMC_ACCObjDstLvl_enum] -> VVMC_ACCObjDstLvl_enum/1
  [VVMC_LKAHODSoundWarning_flg] -> VVMC_LKAHODSoundWarning_flg/1
  [VVMC_ADASCAMSpdLim_enum] -> VVMC_ADASCAMSpdLim_enum/1
  [VVMC_ADASWarningMsg_enum] -> VVMC_ADASWarningMsg_enum/1
  [VVMC_ADASSLIFSpdLim_enum] -> VVMC_ADASSLIFSpdLim_enum/1
  [VVMC_LKAHODDisplayWarning_flg] -> VVMC_LKAHODDisplayWarning_flg/1
  [VVMC_TargetType_enum] -> VVMC_TargetType_enum/1
  [VVMC_ADASLFCSta_enum] -> VVMC_ADASLFCSta_enum/1
  [VVMC_ADASISASta_enum] -> VVMC_ADASISASta_enum/1
  [VVMC_ADASLDWMute_flg] -> VVMC_ADASLDWMute_flg/1
  [VVMC_ADASFCWMute_flg] -> VVMC_ADASFCWMute_flg/1
  [VVMC_ADASSLIFSta_enum] -> VVMC_ADASSLIFSta_enum/1
  [VVMC_ADASLaneModeR_enum] -> VVMC_ADASLaneModeR_enum/1
  [VVMC_ADASLaneModeL_enum] -> VVMC_ADASLaneModeL_enum/1
  [VVMC_ADASLFCHandsOffWarning_enum] -> VVMC_ADASLFCHandsOffWarning_enum/1
  [VVMC_LVDADisabled_flg] -> VVMC_LVDADisabled_flg/1
  [VVMC_LVDAMuteSta_enum] -> VVMC_LVDAMuteSta_enum/1
  [VVMC_LVDAFailinfo_flg] -> VVMC_LVDAFailinfo_flg/1
  [VVMC_LVDAACCStatusInformation_flg] -> VVMC_LVDAACCStatusInformation_flg/1
  [VVMC_LVDAWarning_flg] -> VVMC_LVDAWarning_flg/1
  [VVMC_FCMACCmode_enum] -> VVMC_FCMACCmode_enum/1
  [VVMC_ADASLanetypeR_enum] -> VVMC_ADASLanetypeR_enum/1
  [VVMC_ADASLanecurveR_raw32] -> VVMC_ADASLanecurveR_raw32/1
  [VVMC_ADASLanetypeL_enum] -> VVMC_ADASLanetypeL_enum/1
  [VVMC_ADASLFCWarnSound_enum] -> VVMC_ADASLFCWarnSound_enum/1
  [VVMC_ADASLanecurveL_raw32] -> VVMC_ADASLanecurveL_raw32/1
  [VVMC_ADASAEBReq_enum] -> VVMC_ADASAEBReq_enum/1
  [VVMC_FCMLDWRequest_enum] -> VVMC_FCMLDWRequest_enum/1
  [VVMC_FCMLDWFault_flg] -> VVMC_FCMLDWFault_flg/1
  [VVMC_ADASNegReq_flg] -> VVMC_ADASNegReq_flg/1
  [VVMC_ACCPedalOvrd_flg] -> VVMC_ACCPedalOvrd_flg/1
  [VVMC_ADASWhlTqReq_Nm] -> VVMC_ADASWhlTqReq_Nm/1
  [VVMC_AccPedalOvrdDISC_flg] -> VVMC_AccPedalOvrdDISC_flg/1
  [VVMC_RearTqRatio_rat] -> VVMC_RearTqRatio_rat/1
  [VVMC_TimeGapCalcu_s] -> VVMC_TimeGapCalcu_s/1
  [VVMC_CruzActive_flg] -> VVMC_CruzActive_flg/1
  [VVMC_CruzWhlTqReq_Nm] -> VVMC_CruzWhlTqReq_Nm/1  "VVMC_CruzWhlTqReq_Nm"
  [VVMC_CCCtrlSta_enum] -> VVMC_CCCtrlSta_enum/1
  [VVMC_CCPedalOvrd_flg] -> VVMC_CCPedalOvrd_flg/1  "VVMC_CCPedalOvrd_flg"
  [VVMC_MSAWhlTqReq_Nm] -> VVMC_MSAWhlTqReq_Nm/1
  [VVMC_MSACtrlSta_enum] -> VVMC_MSACtrlSta_enum/1
  [VVMC_MSAActive_flg] -> VVMC_MSAActive_flg/1
  [VVMC_APSDecReq_mps2] -> VVMC_APSDecReq_mps2/1
  [VVMC_APSReq_enum] -> VVMC_APSReq_enum/1
  [VVMC_APSStaSys_enum] -> VVMC_APSStaSys_enum/1
  [VVMC_APSDecReqA_flg] -> VVMC_APSDecReqA_flg/1
  [VVMC_LongAcc_Gps] -> VVMC_LongAcc_Gps/1  "VVMC_LongAcc_Gps"
  [VVMC_RFWhlSpdSlideRate_pct] -> VVMC_RFWhlSpdSlideRate_pct/1
  [VVMC_LRWhlSpdSlideRate_pct] -> VVMC_LRWhlSpdSlideRate_pct/1
  [VVMC_RRWhlSpdSlideRate_pct] -> VVMC_RRWhlSpdSlideRate_pct/1
  [VVMC_RawWhlSpdSlideRate_pct] -> VVMC_RawWhlSpdSlideRate_pct/1
  [VVMC_LFWhlSpdSlideRate_pct] -> VVMC_LFWhlSpdSlideRate_pct/1
  [VVMC_4WhlSpdSlideRate_pct] -> VVMC_4WhlSpdSlideRate_pct/1
  [VVMC_ActRFSlideRate_pct] -> VVMC_ActRFSlideRate_pct/1  "VVMC_ActRFSlideRate_pct"
  [VVMC_LR4WhlSpdSlideRate_pct] -> VVMC_LR4WhlSpdSlideRate_pct/1
  [VVMC_LF4WhlSpdSlideRate_pct] -> VVMC_LF4WhlSpdSlideRate_pct/1
  [VVMC_ActMaxSlideRate_pct] -> VVMC_ActMaxSlideRate_pct/1  "VVMC_ActMaxSlideRate_pct"
  [VVMC_PredictVehSpd_kph] -> VVMC_PredictVehSpd_kph/1
  [VVMC_RF4WhlSpdSlideRate_pct] -> VVMC_RF4WhlSpdSlideRate_pct/1
  [VVMC_ActLFSlideRate_pct] -> VVMC_ActLFSlideRate_pct/1  "VVMC_ActLFSlideRate_pct"
  [VVMC_ActLRSlideRate_pct] -> VVMC_ActLRSlideRate_pct/1  "VVMC_ActLRSlideRate_pct"
  [VVMC_RR4WhlSpdSlideRate_pct] -> VVMC_RR4WhlSpdSlideRate_pct/1
  [VVMC_AltLWhlSlideRate_pct] -> VVMC_AltLWhlSlideRate_pct/1
  [VVMC_ActRRSlideRate_pct] -> VVMC_ActRRSlideRate_pct/1  "VVMC_ActRRSlideRate_pct"
  [VVMC_AltWhlSlideRate_pct] -> VVMC_AltWhlSlideRate_pct/1
  [VVMC_AltRWhlSlideRate_pct] -> VVMC_AltRWhlSlideRate_pct/1
  [VVMC_CCMSASpdWar_flg] -> VVMC_CCMSASpdWar_flg/1
  [VVMC_ACCVehHoldReqRaw_flg] -> SPD2ACC/14(VVMC_ACCVehHoldReqRaw_flg)
  [VVMC_EstSlope_Deg] -> SPD2ACC/15(VVMC_EstSlope_Deg)
  SPD2ACC/10(VVMC_VehHoldDecCtrlHEnd_flg) -> [VVMC_VehHoldDecCtrlHEnd_flg]
  [VTQR_FrTMTqReq_Nm] -> Unit Delay2/1
  Unit Delay2/1 -> ACC_Function/34(VTQR_FrTMTqReq_Nm)
  VTQR_FrTMTqReq_Nm/1 -> [VTQR_FrTMTqReq_Nm]
  VTQD_FrEDUAvailBrkRgnTq_Nm/1 -> [VTQD_FrEDUAvailBrkRgnTq_Nm]
  [VTQD_FrEDUAvailBrkRgnTq_Nm] -> SPD2ACC/16(VTQD_FrEDUAvailBrkRgnTq_Nm)
  [VTQD_RrEDUAvailBrkRgnTq_Nm] -> ACC_Function/35(VTQD_RrEDUAvailBrkRgnTq_Nm)  "VTQD_RrEDUAvailBrkRgnTq_Nm"
  [VTQD_FrEDUAvailBrkRgnTq_Nm] -> ACC_Function/36(VTQD_FrEDUAvailBrkRgnTq_Nm)
  ACC_Function/9(VVMC_ACCLowSpdTqCtrl_flg) -> [VVMC_ACCLowSpdTqCtrl_flg]
  [VVMC_ACCLowSpdTqCtrl_flg] -> SPD2ACC/17(VVMC_ACCLowSpdTqCtrl_flg)
  [VVMC_SafetyCtrl_flg] -> CruiseControlFunction/16(VVMC_SafetyCtrl_flg)
  [VTQR_FrTMTqReq_Nm] -> Unit Delay5/1
  [VTQR_RrTMTqReq_Nm] -> Unit Delay6/1
  [VTQD_RegenMode_enum] -> CruiseControlFunction/19(VTQD_RegenMode_enum)
  [task_time_s] -> CruiseControlFunction/21(task_time_s)
  [VVMC_ActACCRequiredAccel_mps2] -> CruiseControlFunction/20(VVMC_ActACCRequiredAccel_mps2)
  VINP_SASAngle_Deg/1 -> [VINP_SASAngle_Deg]
  <VPMM_DrivetrainSelect_enum>/1 -> [VPMM_DrivetrainSelect_enum]
  [VPMM_DrivetrainSelect_enum] -> ACC_Function/37(VPMM_DrivetrainSelect_enum)
  VMC_FCM1/9(VVMC_ACCVehHoldReqRaw_flg) -> [VVMC_ACCVehHoldReqRaw_flg]  "VVMC_ACCVehHoldReqRaw_flg"
  VMC_FCM1/11(VVMC_ADASACCSta_enum) -> [VVMC_ADASACCSta_enum]  "VVMC_ADASACCSta_enum"
  [VVMC_ActACCRequiredAccel_mps2] -> MSA function/15(VVMC_ActACCRequiredAccel_mps2)
  [VTQR_FrTMTqReq_Nm] -> Unit Delay7/1
  [VTQR_RrTMTqReq_Nm] -> Unit Delay8/1
  Unit Delay5/1 -> CruiseControlFunction/17(VTQR_FrTMTqReq_Nm)
  Unit Delay6/1 -> CruiseControlFunction/18(VTQR_RrTMTqReq_Nm)
  Unit Delay7/1 -> MSA function/16(VTQR_FrTMTqReq_Nm)
  Unit Delay8/1 -> MSA function/17(VTQR_RrTMTqReq_Nm)
  [VINP_Distanceunit_flg] -> FeatureSetSpeed/5(VINP_Distanceunit_flg)  "VINP_Distanceunit_flg"
  Switch5/1 -> Cast To Single34/1
  VTQD_ExtDoorAllow_flg/1 -> [VTQD_ExtDoorAllow_flg]
  Bus Selector10/11 -> IMU/11(VINP_SensingAccY_raw16)  "<VINP_SensingAccY_raw16>"
  IMU/1(VVMC_IMUEnaCmd_flg) -> [VVMC_IMUEnaCmd_flg]
  Bus Selector10/9 -> IMU/9(VINP_SensingGyroZ_raw16)  "<VINP_SensingGyroZ_raw16>"
  Bus Selector10/12 -> IMU/12(VINP_SensingAccZ_raw16)  "<VINP_SensingAccZ_raw16>"
  Bus Selector10/1 -> IMU/1(VINP_MemOffsetGyroX_raw16)  "<VINP_MemOffsetGyroX_raw16>"
  Bus Selector10/2 -> IMU/2(VINP_MemOffsetGyroY_raw16)  "<VINP_MemOffsetGyroY_raw16>"
  Bus Selector10/8 -> IMU/8(VINP_SensingGyroY_raw16)  "<VINP_SensingGyroY_raw16>"
  Bus Selector10/3 -> IMU/3(VINP_MemOffsetGyroZ_raw16)  "<VINP_MemOffsetGyroZ_raw16>"
  [BINP_IMU_outputs] -> Bus Selector10/1
  Bus Selector10/7 -> IMU/7(VINP_SensingGyroX_raw16)  "<VINP_SensingGyroX_raw16>"
  Bus Selector10/4 -> IMU/4(VINP_MemOffsetAccX_raw16)  "<VINP_MemOffsetAccX_raw16>"
  Bus Selector10/6 -> IMU/6(VINP_MemOffsetAccZ_raw16)  "<VINP_MemOffsetAccZ_raw16>"
  Bus Selector10/10 -> IMU/10(VINP_SensingAccX_raw16)  "<VINP_SensingAccX_raw16>"
  Bus Selector10/5 -> IMU/5(VINP_MemOffsetAccY_raw16)  "<VINP_MemOffsetAccY_raw16>"
  VINP_ESCActive_flg/1 -> [VINP_ESCActive_flg]
  VINP_YawRate_degps/1 -> [VINP_YawRate_degps]
  VINP_RDCActive_enum/1 -> [VINP_RDCActive_enum]
  [VVMC_RWDRDCActive_enum] -> VVMC_RWDRDCActive_enum/1
  [VVMC_IMUEnaCmd_flg] -> VVMC_IMUEnaCmd_flg/1
  MSA function/5(VVMC_MSAWhlTqActive_flg) -> [VVMC_MSAWhlTqActive_flg]
  [VVMC_MSAWhlTqActive_flg] -> VVMC_MSAWhlTqActive_flg/1
  VDSC_TurningSpdMovingflat_kph/1 -> [VDSC_TurningSpdMovingflat_kph]
  VDSC_AutoTurnMode_flg/1 -> [VDSC_AutoTurnMode_flg]
  VDSC_AccDecResp_flg/1 -> [VDSC_AccDecResp_flg]
  [VDSC_AutoTurnMode_flg] -> Switch4/2
  Constant7/1 -> Switch4/1
  Switch4/1 -> Cast To Single31/1
  [VDSC_AutoTurnMode_flg] -> Switch5/2
  Constant109/1 -> Switch5/1
  [VDSC_AccDecResp_flg] -> SpeedArbitration/16(VDSC_AccDecResp_flg)
  [task_time_s] -> IMU/13(task_time_s)  "task_time_s"
  [VINP_GRADE_Deg] -> SPD2ACC/18(VINP_GRADE_Deg)
  VINP_LRWhlRotDir_enum/1 -> [VINP_LRWhlRotDir_enum]
  VINP_RFWhlRotDir_enum/1 -> [VINP_RFWhlRotDir_enum]
  VINP_LFWhlRotDir_enum/1 -> [VINP_LFWhlRotDir_enum]
  VINP_RRWhlRotDir_enum/1 -> [VINP_RRWhlRotDir_enum]
  [VINP_RRWhlRotDir_enum] -> SPD2ACC/22(VINP_RRWhlRotDir_enum)
  [VINP_RFWhlRotDir_enum] -> SPD2ACC/21(VINP_RFWhlRotDir_enum)
  [VINP_LRWhlRotDir_enum] -> SPD2ACC/20(VINP_LRWhlRotDir_enum)
  [VINP_LFWhlRotDir_enum] -> SPD2ACC/19(VINP_LFWhlRotDir_enum)
  [VVMC_ACCObjDist_m] -> SPD2ACC/23(VVMC_ACCObjDist_m)
  [VINP_MCPressure_bar] -> SPD2ACC/24(VINP_MCPressure_bar)
  BINP_IMU_outputs/1 -> [BINP_IMU_outputs]
  [VVMC_EstSlope_Deg] -> VVMC_EstSlope_Deg/1  "VVMC_EstSlope_Deg"
  Long Acceleration Calculation/2(VVMC_EstSlope_Deg) -> [VVMC_EstSlope_Deg]
  [VTQD_RrEDUAvailBrkRgnTq_Nm] -> Add/2
  [VTQD_FrEDUAvailBrkRgnTq_Nm] -> Add/1
  Add/1 -> [VVMC_TotalAvailBrkRgnTq_Nm]
  [VVMC_TotalAvailBrkRgnTq_Nm] -> ACC_Function/38(VVMC_TotalAvailBrkRgnTq_Nm)
  [VVMC_TotalAvailBrkRgnTq_Nm] -> CruiseControlFunction/22(VVMC_TotalAvailBrkRgnTq_Nm)
  [VVMC_TotalAvailBrkRgnTq_Nm] -> MSA function/18(VVMC_TotalAvailBrkRgnTq_Nm)
  [VVMC_AccelTurnHold_flg] -> ACC_Function/39(VVMC_AccelTurnHold_flg)
  [VVMC_ADASACCSta_enum] -> ACC_Function/40(VVMC_ADASACCSta_enum)
  [VDSC_AutoTurnMode_flg] -> SpeedArbitration/17(VDSC_AutoTurnMode_flg)
  [VTQD_GearActualPosn_enum] -> Slide Rate  Calculation/14(VTQD_GearActualPosn_enum)
  [VTQD_EquivAccPedalSWSta_flg] -> Slide Rate  Calculation/13(VTQD_EquivAccPedalSWSta_flg)
  [VTQD_AfterAvailableTqDemRr_Nm] -> Slide Rate  Calculation/12(VTQD_AfterAvailableTqDemRr_Nm)
  [VTQD_AfterAvailableTqDemFr_Nm] -> Slide Rate  Calculation/11(VTQD_AfterAvailableTqDemFr_Nm)
  [task_time_s] -> Slide Rate  Calculation/10(task_time_s)  "task_time_s"
  [VINP_BrkSwSta_flg] -> Slide Rate  Calculation/7(VINP_BrkSwSta_flg)
  [VINP_BrkPedalPos_pct] -> Slide Rate  Calculation/6(VINP_BrkPedalPos_pct)
  [VINP_VehSpeed_kph] -> Slide Rate  Calculation/5(VINP_VehSpeed_kph)
  [VINP_RRRawWhlSpeed_kph] -> Slide Rate  Calculation/4(VINP_RRRawWhlSpeed_kph)
  [VINP_LRRawWhlSpeed_kph] -> Slide Rate  Calculation/3(VINP_LRRawWhlSpeed_kph)
  [VINP_RFRawWhlSpeed_kph] -> Slide Rate  Calculation/2(VINP_RFRawWhlSpeed_kph)
  [VINP_LFRawWhlSpeed_kph] -> Slide Rate  Calculation/1(VINP_LFRawWhlSpeed_kph)
  Switch8/1 -> Slide Rate  Calculation/8(VINP_LongAccel_Gps)
  [VVMC_LongAcc_Gps] -> Slide Rate  Calculation/9(VVMC_LongAcc_Gps)  "VVMC_LongAcc_Gps"
  Slide Rate  Calculation/1(VVMC_RawWhlSpdSlideRate_pct) -> [VVMC_RawWhlSpdSlideRate_pct]
  Slide Rate  Calculation/2(VVMC_LFWhlSpdSlideRate_pct) -> [VVMC_LFWhlSpdSlideRate_pct]
  Slide Rate  Calculation/3(VVMC_RFWhlSpdSlideRate_pct) -> [VVMC_RFWhlSpdSlideRate_pct]
  Slide Rate  Calculation/4(VVMC_LRWhlSpdSlideRate_pct) -> [VVMC_LRWhlSpdSlideRate_pct]
  Slide Rate  Calculation/5(VVMC_RRWhlSpdSlideRate_pct) -> [VVMC_RRWhlSpdSlideRate_pct]
  Slide Rate  Calculation/6(VVMC_LF4WhlSpdSlideRate_pct) -> [VVMC_LF4WhlSpdSlideRate_pct]
  Slide Rate  Calculation/7(VVMC_RF4WhlSpdSlideRate_pct) -> [VVMC_RF4WhlSpdSlideRate_pct]
  Slide Rate  Calculation/8(VVMC_LR4WhlSpdSlideRate_pct) -> [VVMC_LR4WhlSpdSlideRate_pct]
  Slide Rate  Calculation/9(VVMC_RR4WhlSpdSlideRate_pct) -> [VVMC_RR4WhlSpdSlideRate_pct]
  Slide Rate  Calculation/10(VVMC_PredictVehSpd_kph) -> [VVMC_PredictVehSpd_kph]
  Slide Rate  Calculation/11(VVMC_4WhlSpdSlideRate_pct) -> [VVMC_4WhlSpdSlideRate_pct]
  Slide Rate  Calculation/12(VVMC_ActMaxSlideRate_pct) -> [VVMC_ActMaxSlideRate_pct]
  Slide Rate  Calculation/13(VVMC_ActLFSlideRate_pct) -> [VVMC_ActLFSlideRate_pct]
  Slide Rate  Calculation/14(VVMC_ActRFSlideRate_pct) -> [VVMC_ActRFSlideRate_pct]
  Slide Rate  Calculation/15(VVMC_ActLRSlideRate_pct) -> [VVMC_ActLRSlideRate_pct]
  Slide Rate  Calculation/16(VVMC_ActRRSlideRate_pct) -> [VVMC_ActRRSlideRate_pct]
  Slide Rate  Calculation/17(VVMC_AltLWhlSlideRate_pct) -> [VVMC_AltLWhlSlideRate_pct]
  Slide Rate  Calculation/18(VVMC_AltRWhlSlideRate_pct) -> [VVMC_AltRWhlSlideRate_pct]
  Slide Rate  Calculation/19(VVMC_AltWhlSlideRate_pct) -> [VVMC_AltWhlSlideRate_pct]
  [task_time_s] -> RDC Determination/1(task_time_s)  "task_time_s"
  [VVMC_ActMaxSlideRate_pct] -> RDC Determination/2(VVMC_ActMaxSlideRate_pct)
  [VTQD_AfterAvailableTqDemFr_Nm] -> RDC Determination/3(VTQD_AfterAvailableTqDemFr_Nm)
  [VTQD_AfterAvailableTqDemRr_Nm] -> RDC Determination/4(VTQD_AfterAvailableTqDemRr_Nm)
  [VINP_ESCActive_flg] -> RDC Determination/5(VINP_ESCActive_flg)
  [VINP_SASAngle_Deg] -> RDC Determination/6(VINP_SASAngle_Deg)
  Switch6/1 -> RDC Determination/7(VINP_LatAccel_Gps)
  [VINP_VehSpeed_kph] -> RDC Determination/8(VINP_VehSpeed_kph)
  Switch7/1 -> RDC Determination/9(VINP_YawRate_degps)
  [VINP_RDCActive_enum] -> RDC Determination/10(VINP_RDCActive_enum)
  RDC Determination/1(VVMC_RWDRDCActive_enum) -> [VVMC_RWDRDCActive_enum]
  RDC Determination/2(VVMC_RDCEnSlideRate_pct) -> [VVMC_RDCEnSlideRate_pct]
  RDC Determination/3(VVMC_ActStESCYaw_degps) -> [VVMC_ActStESCYaw_Dps]
  [VVMC_RDCEnSlideRate_pct] -> VVMC_RDCEnSlideRate_pct/1
  [VVMC_ActStESCYaw_Dps] -> VVMC_ActStESCYaw_Dps/1
  [VINP_HoodSW_flg] -> MSA function/19(VINP_HoodSW_flg)
  VINP_HoodSW_flg/1 -> [VINP_HoodSW_flg]
  [VTQD_GearActualPosn_enum] -> MSA function/20(VTQD_GearActualPosn_enum)
  [VVMC_AntiSpdLimSpdEn_flg] -> SpeedArbitration/18(VVMC_AntiSpdLimSpdEn_flg)
  [VTQD_ExtDoorAllow_flg] -> ACC_Function/41(VTQD_ExtDoorAllow_flg)
  VINP_DIDGetDynoMode_flg/1 -> [VINP_DIDGetDynoMode_flg]
  [VINP_DIDGetDynoMode_flg] -> RDC Determination/11(VINP_DIDGetDynoMode_flg)
  [VINP_DIDGetDynoMode_flg] -> Long Acceleration Calculation/8(VINP_DIDGetDynoMode_flg)
  [VINP_SASAngle_Deg] -> ACC_Function/42(VINP_SASAngle_Deg)
  [VINP_Distanceunit_flg] -> CruiseControlFunction/23(VINP_Distanceunit_flg)
  [VINP_Distanceunit_flg] -> MSA function/21(VINP_Distanceunit_flg)
  IMU/2(VVMC_CalibratedGyroX_Dps) -> [VVMC_CalibratedGyroX_Dps]
  IMU/3(VVMC_CalibratedGyroY_Dps) -> [VVMC_CalibratedGyroY_Dps]
  IMU/4(VVMC_CalibratedGyroZ_Dps) -> [VVMC_CalibratedGyroZ_Dps]
  IMU/5(VVMC_CalibratedAccX_G) -> [VVMC_CalibratedAccX_G]
  IMU/6(VVMC_CalibratedAccY_G) -> [VVMC_CalibratedAccY_G]
  IMU/7(VVMC_CalibratedAccZ_G) -> [VVMC_CalibratedAccZ_G]
  [VDHP_ActAPSPosn_pct] -> ACC_Function/43(VDHP_ActAPSPosn_pct)
  Constant28/1 -> AND4/2
  [VVMC_IMUEnaCmd_flg] -> AND4/1
  [VVMC_CalibratedAccY_G] -> Switch6/1
  AND4/1 -> Switch6/2
  [VINP_LatAccel_Gps] -> Switch6/3
  AND5/1 -> Switch7/2
  [VVMC_CalibratedGyroZ_Dps] -> Switch7/1
  [VVMC_IMUEnaCmd_flg] -> AND5/1
  Constant10/1 -> AND5/2
  [VINP_YawRate_degps] -> Switch7/3
  AND6/1 -> Switch8/2
  [VVMC_IMUEnaCmd_flg] -> AND6/1
  Constant11/1 -> AND6/2
  [VVMC_CalibratedAccX_G] -> Switch8/1
  [VINP_LongAccel_Gps] -> Switch8/3
  VTQD_CreepBaseTqD_Nm/1 -> [VTQD_CreepBaseTqD_Nm]
  [VTQD_CreepBaseTqD_Nm] -> ACC_Function/44(VTQD_CreepBaseTqD_Nm)
  ACC_Function/10(VVMC_ACCOvrdMemTq_Nm) -> [VVMC_ACCOvrdMemTq_Nm]
  [VVMC_ACCOvrdMemTq_Nm] -> VVMC_ACCOvrdMemTq_Nm/1
  [VVMC_EstSlope_Deg] -> Slide Rate  Calculation/17(VVMC_EstSlope_Deg)
  [VTQD_VehActSpd_kph] -> Slide Rate  Calculation/16(VTQD_VehActSpd_kph)
  [VTQD_RegenMode_enum] -> Slide Rate  Calculation/15(VTQD_RegenMode_enum)
  VTQD_VehActSpd_kph/1 -> [VTQD_VehActSpd_kph]
  APS function/1(VVMC_APSCtrlAvail_flg) -> [VVMC_APSCtrlAvail_flg]
  APS function/2(VVMC_APSActive_flg) -> [VVMC_APSActive_flg]
  APS function/3(VVMC_CAASCtrlAvail_flg) -> [VVMC_CAASCtrlAvail_flg]
  APS function/10(VVMC_APSReq_enum) -> [VVMC_APSReq_enum]
  APS function/9(VVMC_APSDecReq_mps2) -> [VVMC_APSDecReq_mps2]
  APS function/8(VVMC_APSDecReqA_flg) -> [VVMC_APSDecReqA_flg]
  APS function/7(VVMC_APSStaSys_enum) -> [VVMC_APSStaSys_enum]
  APS function/6(VVMC_APSShiftPosnReq_enum) -> [VVMC_APSShiftPosnReq_enum]
  APS function/5(VVMC_APSSpeedCMD_kph) -> [VVMC_APSSpeedCMD_kph]
  APS function/4(VVMC_CAASActive_flg) -> [VVMC_CAASActive_flg]
  [VVMC_CAASCtrlAvail_flg] -> VVMC_CAASCtrlAvail_flg/1
  [VVMC_CAASActive_flg] -> VVMC_CAASActive_flg/1
  [VVMC_CalibratedGyroY_Dps] -> VVMC_CalibratedGyroY_Dps/1  "VVMC_CalibratedGyroY_Dps"
  VINP_APSStaSystem_enum/1 -> [VINP_APSStaSystem_enum]
  VINP_CAASVMCReqA_flg/1 -> [VINP_CAASVMCReqA_flg]
  VINP_APSReq_enum/1 -> [VINP_APSReq_enum]
  VINP_APSDecReq_mps2/1 -> [VINP_APSDecReq_mps2]
  VINP_APSDecReqA_flg/1 -> [VINP_APSDecReqA_flg]
  MSA function/6(VVMC_ExtraMSACtrlSta_enum) -> [VVMC_ExtraMSACtrlSta_enum]
  [VVMC_ExtraMSACtrlSta_enum] -> "VVMC_ExtraMSACtrlSta_enum "/1
  [VVMC_CalibratedGyroX_Dps] -> VVMC_CalibratedGyroX_Dps/1  "VVMC_CalibratedGyroX_Dps"
  [VVMC_CalibratedGyroZ_Dps] -> VVMC_CalibratedGyroZ_Dps/1  "VVMC_CalibratedGyroZ_Dps"
  [VVMC_CalibratedAccX_G] -> VVMC_CalibratedAccX_G/1  "VVMC_CalibratedAccX_G"
  [VVMC_CalibratedAccY_G] -> VVMC_CalibratedAccY_G/1  "VVMC_CalibratedAccY_G"
  [VVMC_CalibratedAccZ_G] -> VVMC_CalibratedAccZ_G/1  "VVMC_CalibratedAccZ_G"
  VINP_IVISWCVibModeSta_enum/1 -> [VINP_IVISWCVibModeSta_enum]
  APS function/11(VVMC_SetACCDisableAPS_flg) -> [VVMC_SetACCDisableAPS_flg]
  [VVMC_SetACCDisableAPS_flg] -> VVMC_SetACCDisableAPS_flg/1
  VINP_SmartEcoModeSW_flg/1 -> [VINP_SmartEcoModeSW_flg]
  [VINP_SmartEcoModeSW_flg] -> MSA function/22(VINP_SmartEcoModeSW_flg)
  [VVMC_APSActive_flg] -> MSA function/23(VVMC_APSActive_flg)
  MSA function/7(VVMC_AntiLimitSpd_kph) -> [VVMC_AntiLimitSpd_kph]
  MSA function/8(VVMC_AntiSpdLimSpdEn_flg) -> [VVMC_AntiSpdLimSpdEn_flg]
  [VVMC_AntiLimitSpd_kph] -> SpeedArbitration/19(VVMC_AntiLimitSpd_kph)
  [VTQD_ExtDoorAllow_flg] -> CruiseControlFunction/24(VTQD_ExtDoorAllow_flg)
  [VVMC_ACCShutOffHold_flg] -> VMC_FCM1/58(VVMC_ACCShutOffHold_flg)
  [VVMC_ACCShutOffHold_flg] -> ACC_Function/45(VVMC_ACCShutOffHold_flg)
  [VINP_ADASACCSta_enum] -> ACC_Function/46(VINP_ADASACCSta_enum)
  [VVMC_VMCCCCtrlAvail_flg] -> CruiseControlFunction/25(VVMC_VMCCCCtrlAvail_flg)
  [VVMC_VMCMSACtrlAvail_flg] -> MSA function/24(VVMC_VMCMSACtrlAvail_flg)
  VINP_APSShiftPosnReq_enum/1 -> [VINP_APSShiftPosnReq_enum]
  VINP_APSVMCReqA_flg/1 -> [VINP_APSVMCReqA_flg]
  VDSC_PreACC_mps2/1 -> [VDSC_PreACC_mps2]
  VDSC_PreACC_flg/1 -> [VDSC_PreACC_flg]
  [VDSC_AutoTurnMode_flg] -> AND9/1
  AND9/1 -> Switch2/2
  Constant15/1 -> Relational Operator8/2
  Relational Operator8/1 -> AND9/2
  [VDSC_DISCTargetSpd_kph] -> Switch2/3  "VDSC_DISCTargetSpd_kph"
  [VDSC_DISCSta_enum] -> Relational Operator8/1
  [VDSC_TurningSpdMovingflat_kph] -> Switch2/1
  [VDSC_AccDecResp_flg] -> SPD2ACC/29(VDSC_AccDecResp_flg)
  [VDSC_AutoTurnMode_flg] -> SPD2ACC/28(VDSC_AutoTurnMode_flg)
  [VDSC_PreACC_flg] -> SPD2ACC/25(VDSC_PreACC_flg)
  [VDSC_PreACC_mps2] -> SPD2ACC/26(VDSC_PreACC_mps2)
  [VDSC_DISCSta_enum] -> SPD2ACC/27(VDSC_DISCSta_enum)
  [VDSC_PreACC_flg] -> SpeedArbitration/20(VDSC_PreACC_flg)
  SPD2ACC/11(VVMC_AccelTurnHold_flg) -> [VVMC_AccelTurnHold_flg]
  SPD2ACC/12(VVMC_ACCVehHoldReq_flg) -> [VVMC_ACCVehHoldReq_flg]
  SPD2ACC/13(VVMC_ACCShutOffHold_flg) -> [VVMC_ACCShutOffHold_flg]
  [VINP_BrkSwSta_flg] -> SPD2ACC/30(VINP_BrkSwSta_flg)
  [VINP_ACCVehHoldReq_flg] -> SPD2ACC/31(VINP_ACCVehHoldReq_flg)
  [VTQD_GearActualPosn_enum] -> SPD2ACC/32(VTQD_GearActualPosn_enum)
  [VTQD_LowIdleAccPedal_flg] -> SPD2ACC/33(VTQD_LowIdleAccPedal_flg)
  [VINP_EPBSta_enum] -> SPD2ACC/34(VINP_EPBSta_enum)
  VINP_FrTMSpdNidec_rpm/1 -> Switch1/3
  VINP_FrTMSpd_rpm/1 -> Switch1/1
  Switch1/1 -> [VINP_FrTMSpd_rpm]  "VINP_FrTMSpd_rpm"
  Switch3/1 -> [VINP_RrTMSpd_rpm]  "VINP_RrTMSpd_rpm"
  VINP_RrTMSpd_rpm/1 -> Switch3/1
  VINP_ADASDrvInputTqBoostAct_flg/1 -> [VINP_ADASDrvInputTqBoostAct_flg]
  VINP_ADASStrWhlAngCtrlStatus_flg/1 -> [VINP_ADASStrWhlAngCtrlStatus_flg]
  VINP_ADASMaxAngCtrlOutTqLimit_Nm/1 -> [VINP_ADASMaxAngCtrlOutTqLimit_Nm]
  VINP_ADASDrvInputTqBoostGain_pct/1 -> [VINP_ADASDrvInputTqBoostGain_pct]
  VINP_ADASAngCtrlTqWeightGain_pct/1 -> [VINP_ADASAngCtrlTqWeightGain_pct]
  VINP_ADASDesStrWhlAngCtrlCmd_Deg/1 -> [VINP_ADASDesStrWhlAngCtrlCmd_Deg]
  [VVMC_FDCVMCAPSVRqEPSCtrl_flg] -> VVMC_FDCVMCAPSVRqEPSCtrl_flg/1
  [VVMC_FDCVMCAPSRqEPSCtrl_flg] -> VVMC_FDCVMCAPSRqEPSCtrl_flg/1
  [VVMC_FDCVMCAPSAngleTarget_deg] -> VVMC_FDCVMCAPSAngleTarget_deg/1
  VINP_APSAngleTarget_Deg/1 -> [VINP_APSAngleTarget_Deg]
  VINP_APSRqEPASCtrl_flg/1 -> [VINP_APSRqEPASCtrl_flg]
  VINP_APSVRqEPASCtrl_flg/1 -> [VINP_APSVRqEPASCtrl_flg]
  [VVMC_FDCVMCDrInpTqBstGn_pct] -> VVMC_FDCVMCDrInpTqBstGn_pct/1  "VVMC_FDCVMCDrInpTqBstGn_pct"
  [VVMC_FDCVMCMaxAngCtrlOutTqLim_Nm] -> VVMC_FDCVMCMaxAngCtrlOutTqLim_Nm/1  "VVMC_FDCVMCMaxAngCtrlOutTqLim_Nm"
  [VVMC_FDCVMCDrInpTqBstAct_flg] -> VVMC_FDCVMCDrInpTqBstAct_flg/1  "VVMC_FDCVMCDrInpTqBstAct_flg"
  [VVMC_FDCVMCAngCtrlTqWtGn_pct] -> VVMC_FDCVMCAngCtrlTqWtGn_pct/1
  [VINP_VehicleType_enum] -> Equal1/1
  Constant14/1 -> Equal1/2
  Equal1/1 -> Switch1/2
  Constant6/1 -> Equal2/2
  [VINP_VehicleType_enum] -> Equal2/1
  Equal2/1 -> Switch3/2
  VINP_SWCType_enum/1 -> [VINP_SWCType_enum]
  VINP_VehicleType_enum/1 -> [VINP_VehicleType_enum]
  [VINP_SWCType_enum] -> MSA function/25(VINP_SWCType_enum)
  VTQD_EVDriveMode_enum/1 -> [VTQD_EVDriveMode_enum]
  [VTQD_EVDriveMode_enum] -> ACC_Function/47(VTQD_EVDriveMode_enum)
  VTQD_SWC1CANCELSta_flg/1 -> [VTQD_SWC1CANCELSta_flg]
  VTQD_SWC1ResUpSta_flg/1 -> [VTQD_SWC1ResUpSta_flg]
  VTQD_SWC1SetdownSta_flg/1 -> [VTQD_SWC1SetdownSta_flg]
  [VTQD_SWC1CANCELSta_flg] -> MSA function/26(VTQD_SWC1CANCELSta_flg)
  [VTQD_SWC1ResUpSta_flg] -> MSA function/27(VTQD_SWC1ResUpSta_flg)
  [VTQD_SWC1SetdownSta_flg] -> MSA function/28(VTQD_SWC1SetdownSta_flg)
  [VINP_APSVRqEPASCtrl_flg] -> LFCAOIControl/1(VINP_APSVRqEPASCtrl_flg)
  [VINP_ADASDrvInputTqBoostAct_flg] -> LFCAOIControl/7(VINP_ADASDrvInputTqBoostAct_flg)
  [VINP_APSRqEPASCtrl_flg] -> LFCAOIControl/2(VINP_APSRqEPASCtrl_flg)
  [VINP_ADASStrWhlAngCtrlStatus_flg] -> LFCAOIControl/3(VINP_ADASStrWhlAngCtrlStatus_flg)
  [VINP_APSAngleTarget_Deg] -> LFCAOIControl/4(VINP_APSAngleTarget_Deg)
  [VINP_ADASDesStrWhlAngCtrlCmd_Deg] -> LFCAOIControl/5(VINP_ADASDesStrWhlAngCtrlCmd_Deg)
  [VINP_ADASMaxAngCtrlOutTqLimit_Nm] -> LFCAOIControl/8(VINP_ADASMaxAngCtrlOutTqLimit_Nm)
  [VINP_ADASDrvInputTqBoostGain_pct] -> LFCAOIControl/9(VINP_ADASDrvInputTqBoostGain_pct)
  [VINP_VehicleType_enum] -> LFCAOIControl/10(VINP_VehicleType_enum)
  [VINP_ADASAngCtrlTqWeightGain_pct] -> LFCAOIControl/6(VINP_ADASAngCtrlTqWeightGain_pct)
  LFCAOIControl/6(VVMC_FDCVMCMaxAngCtrlOutTqLim_Nm) -> [VVMC_FDCVMCMaxAngCtrlOutTqLim_Nm]
  LFCAOIControl/1(VVMC_FDCVMCAPSVRqEPSCtrl_flg) -> [VVMC_FDCVMCAPSVRqEPSCtrl_flg]
  LFCAOIControl/2(VVMC_FDCVMCAPSRqEPSCtrl_flg) -> [VVMC_FDCVMCAPSRqEPSCtrl_flg]
  LFCAOIControl/3(VVMC_FDCVMCAPSAngleTarget_deg) -> [VVMC_FDCVMCAPSAngleTarget_deg]
  LFCAOIControl/4(VVMC_FDCVMCAngCtrlTqWtGn_pct) -> [VVMC_FDCVMCAngCtrlTqWtGn_pct]
  LFCAOIControl/5(VVMC_FDCVMCDrInpTqBstAct_flg) -> [VVMC_FDCVMCDrInpTqBstAct_flg]
  LFCAOIControl/7(VVMC_FDCVMCDrInpTqBstGn_pct) -> [VVMC_FDCVMCDrInpTqBstGn_pct]
  VDDM_VMCEPSErr_flg/1 -> [VDDM_VMCEPSErr_flg]
  VDDM_VMCESC5Err_flg/1 -> [VDDM_VMCESC5Err_flg]
  VDDM_VMCESC1Err_flg/1 -> [VDDM_VMCESC1Err_flg]
  VDDM_VMCLatCtrlProhibited_flg/1 -> [VDDM_VMCLatCtrlProhibited_flg]
  VDDM_VMCLongCtrlProhibited_flg/1 -> [VDDM_VMCLongCtrlProhibited_flg]
  [VDDM_VMCLongCtrlProhibited_flg] -> PreConditionCheck/12(VDDM_VMCLongCtrlProhibited_flg)
  [VINP_IVISWCVibModeSta_enum] -> VMC_FCM1/59(VINP_IVISWCVibModeSta_enum)
  [VDDM_VMCLatCtrlProhibited_flg] -> VMC_FCM1/60(VDDM_VMCLatCtrlProhibited_flg)
  [VDDM_VMCLongCtrlProhibited_flg] -> VMC_FCM1/61(VDDM_VMCLongCtrlProhibited_flg)
  [VDDM_VMCLatCtrlProhibited_flg] -> LFCAOIControl/11(VDDM_VMCLatCtrlProhibited_flg)
  [VINP_MeterIndVehSpeed_kph] -> SpeedCalculation/1(VINP_MeterIndVehSpeed_kph)  "VINP_METERKPHCalcu_kph"
  [VINP_VehSpeed_kph] -> SpeedCalculation/3(VINP_VehSpeed_kph)
  [VDDM_VMCESC1Err_flg] -> SpeedCalculation/5(VDDM_VMCESC1Err_flg)
  [VDDM_VMCESC5Err_flg] -> SpeedCalculation/6(VDDM_VMCESC5Err_flg)
  [VINP_Distanceunit_flg] -> SpeedCalculation/2(VINP_Distanceunit_flg)  "VINP_Distanceunit_flg"
  [VTQD_VehActSpd_kph] -> SpeedCalculation/4(VTQD_VehActSpd_kph)
  SafetyControl/2(VVMC_FrontRearSlipRatioCtrl_flg) -> [VVMC_FrontRearSlipRatioCtrl_flg]
  SafetyControl/1(VVMC_SafetyCtrl_flg) -> [VVMC_SafetyCtrl_flg]
  SafetyControl/3(VVMC_RearWhlSlipRatioCtrl_flg) -> [VVMC_RearWhlSlipRatioCtrl_flg]
  SafetyControl/4(VVMC_SingleWhlSlipRatioCtrl_flg) -> [VVMC_SingleWhlSlipRatioCtrl_flg]
  SafetyControl/5(VVMC_LatAccCtrl_flg) -> [VVMC_LatAccCtrl_flg]
  SafetyControl/6(VVMC_EstSlope_Deg) -> [VVMC_EstSlopeCal_Deg]
  SafetyControl/7(VVMC_LFWhlSpeedRollAve_kph) -> [VVMC_LFWhlSpeedRollAve_kph]
  SafetyControl/8(VVMC_RFWhlSpeedRollAve_kph) -> [VVMC_RFWhlSpeedRollAve_kph]
  SafetyControl/9(VVMC_LRWhlSpeedRollAve_kph) -> [VVMC_LRWhlSpeedRollAve_kph]
  SafetyControl/10(VVMC_RRWhlSpeedRollAve_kph) -> [VVMC_RRWhlSpeedRollAve_kph]
  SafetyControl/11(VVMC_LongAccelCalcuByVehSpdRaw_gps) -> [VVMC_LongAccelCalcuByVehSpdRaw_gps]
  SafetyControl/12(VVMC_FrRrSlipSpd_kph) -> [VVMC_FrRrSlipSpd_kph]
  initial = 0/1 -> SafetyControl/12(VVMC_FeatArbitrFinal_enum)  "VVMC_FeatArbitrFinal_enum"
  [VDDM_VMCESC1Err_flg] -> SafetyControl/18(VDDM_VMCESC1Err_flg)
  [VDDM_VMCESC5Err_flg] -> SafetyControl/19(VDDM_VMCESC5Err_flg)
  [VVMC_CalibratedAccX_G] -> SafetyControl/15(VVMC_CalibratedAccX_G)
  [VVMC_IMUEnaCmd_flg] -> SafetyControl/16(VVMC_IMUEnaCmd_flg)
  [VTQD_VehActSpd_kph] -> SafetyControl/17(VTQD_VehActSpd_kph)
  [VINP_LFRawWhlSpeed_kph] -> SafetyControl/2(VINP_LFRawWhlSpeed_kph)
  [VINP_LFRawWhlSpeedV_flg] -> SafetyControl/3(VINP_LFRawWhlSpeedV_flg)
  [VINP_RFRawWhlSpeed_kph] -> SafetyControl/4(VINP_RFRawWhlSpeed_kph)
  [VINP_RFRawWhlSpeedV_flg] -> SafetyControl/5(VINP_RFRawWhlSpeedV_flg)
  [VINP_LRRawWhlSpeed_kph] -> SafetyControl/6(VINP_LRRawWhlSpeed_kph)
  [VINP_LRRawWhlSpeedV_flg] -> SafetyControl/7(VINP_LRRawWhlSpeedV_flg)
  [VINP_RRRawWhlSpeed_kph] -> SafetyControl/8(VINP_RRRawWhlSpeed_kph)
  [VINP_RRRawWhlSpeedV_flg] -> SafetyControl/9(VINP_RRRawWhlSpeedV_flg)
  [VINP_LatAccel_Gps] -> SafetyControl/10(VINP_LatAccel_Gps)
  [VINP_LatAccelV_flg] -> SafetyControl/11(VINP_LatAccelV_flg)
  [VINP_LongAccel_Gps] -> SafetyControl/13(VINP_LongAccel_Gps)
  [VINP_GRADE_Deg] -> SafetyControl/14(VINP_GRADE_deg)
  [VINP_VehSpeed_kph] -> SafetyControl/1(VINP_VehSpeed_kph)
  [VDDM_VMCEPSErr_flg] -> LFCAOIControl/12(VDDM_VMCEPSErr_flg)
  SPD2ACC/14(VVMC_OVRD2ActRampActive_flg) -> [VVMC_OVRD2ActRampActive_flg]
  [VVMC_OVRD2ActRampActive_flg] -> ACC_Function/48(VVMC_OVRD2ActRampActive_flg)
  [VINP_ACCRequiredAccel_mps2] -> ACC_Function/49(VINP_ACCRequiredAccel_mps2)  "VINP_ACCRequiredAccel_mps2"
  [VVMC_FeatSetSpdFinal_raw32] -> CruiseControlFunction/26(VVMC_FeatSetSpdFinal_raw32)
  [VVMC_FeatSetSpdFinal_raw32] -> MSA function/29(VVMC_FeatSetSpdFinal_raw32)
  [VTQD_APSReq_enum] -> APS function/14(VTQD_APSReq_enum)
  [VINP_SCPSystemMode_enum] -> APS function/9(VINP_SCPSystemMode_enum)
  [VTQD_ExternalTqAllow_flg] -> APS function/1(VTQD_ExternalTqAllow_flg)  "VTQD_ExternalTqAllow_flg"
  [VINP_APSVMCReqA_flg] -> APS function/5(VINP_APSVMCReqA_flg)  "VAPS_APSVMCReqA_flg"
  [VTQD_APSDecReqA_flg] -> APS function/12(VTQD_APSDecReqA_flg)
  [VINP_APSSpeedCMD_kph] -> APS function/7(VINP_APSSpeedCMD_kph)  "VAPS_APSSpeedCMD_kph"
  [VVMC_ADASActive_flg] -> APS function/10(VVMC_ADASActive_flg)
  [VTQD_APSDecReq_mps2] -> APS function/13(VTQD_APSDecReq_mps2)
  [VINP_APSShiftPosnReq_enum] -> APS function/6(VINP_APSShiftPosnReq_enum)  "VAPS_APSShiftPosnReq_enum"
  [VINP_CAASVMCReqA_flg] -> APS function/21(VINP_CAASVMCReqA_flg)
  [VINP_APSDecReq_mps2] -> APS function/17(VINP_APSDecReq_mps2)
  [VDDM_VCURAPSErrLv2_flg] -> APS function/28(VDDM_VCURAPSErrLv2_flg)
  [VINP_ACCObjDist_m] -> APS function/26(VINP_ACCObjDist_m)
  [VTQD_EPBCarWashMode_flg] -> APS function/30(VTQD_EPBCarWashMode_flg)
  [VTQD_ExtDoorAllow_flg] -> APS function/3(VTQD_ExtDoorAllow_flg)
  [VINP_VehSpeed_kph] -> APS function/19(VINP_VehSpeed_kph)
  [VVMC_MeterIndSpeedForCalcu_kph] -> APS function/27(VVMC_MeterIndSpeedForCalcu_kph)
  [VVMC_CruzActive_flg] -> APS function/20(VVMC_CruzActive_flg)
  [VDDM_VCURAPSErrLv3_flg] -> APS function/29(VDDM_VCURAPSErrLv3_flg)
  [VTQD_GearActualPosn_enum] -> APS function/4(VTQD_GearActualPosn_enum)  "VAPS_APSStaSystem_enum"
  [VINP_MCPressure_bar] -> APS function/24(VINP_MCPressure_bar)
  [task_time_s] -> APS function/8(task_time_s)  "task_time_s"
  [VINP_BrkSwSta_flg] -> APS function/23(VINP_BrkSwSta_flg)
  [VINP_BrkPedalPos_pct] -> APS function/25(VINP_BrkPedalPos_pct)
  [VTQD_ExtShftAllow_flg] -> APS function/2(VTQD_ExtShiftAllow_flg)  "VTQD_ExtShftAllow_flg"
  [VINP_APSDecReqA_flg] -> APS function/16(VINP_APSDecReqA_flg)
  [VINP_APSStaSystem_enum] -> APS function/15(VINP_APSStaSystem_enum)
  [VINP_ADASACCSta_enum] -> APS function/22(VINP_ADASACCSta_enum)
  [VINP_APSReq_enum] -> APS function/18(VINP_APSReq_enum)
  [VTQD_APSStaSys_enum] -> APS function/11(VTQD_APSStaSys_enum)
  VINP_SCPSystemMode_enum/1 -> [VINP_SCPSystemMode_enum]
  VTQD_EPBCarWashMode_flg/1 -> [VTQD_EPBCarWashMode_flg]
  VDDM_VCURAPSErrLv2_flg/1 -> [VDDM_VCURAPSErrLv2_flg]
  VDDM_VCURAPSErrLv3_flg/1 -> [VDDM_VCURAPSErrLv3_flg]
  [VTQD_SWC1ResUpSta_flg] -> ACC_Function/50(VTQD_SWC1ResUpSta_flg)
  [VINP_SWCType_enum] -> ACC_Function/51(VINP_SWCType_enum)
